simulink model "model"  (R2016a)
(part 11 of 11)

  _CN_176704629_220000_CN30425117/RConn3 -- G_30425117_Kraftwerk_Weiher/RConn3 -- _CN_54359256_220000_CN30425117/RConn3 -- _CN_100812630_220000_CN30425117/LConn3
  T_150267232_220000_LMG/LConn1 -- 220kV_LMG_West_CN_24921206_220000_CN_150267232_220000/RConn1
  T_150267232_220000_LMG/LConn2 -- 220kV_LMG_West_CN_24921206_220000_CN_150267232_220000/RConn2
  T_150267232_220000_LMG/LConn3 -- 220kV_LMG_West_CN_24921206_220000_CN_150267232_220000/RConn3
  T_42423415_220000;110000_Station_Meckenheim/LConn1 -- 220_kV_Berggeist_West;_Nette_Ost_CN_42423415_220000_CN_395847307_220000/RConn1
  T_42423415_220000;110000_Station_Meckenheim/LConn2 -- 220_kV_Berggeist_West;_Nette_Ost_CN_42423415_220000_CN_395847307_220000/RConn2
  T_42423415_220000;110000_Station_Meckenheim/LConn3 -- 220_kV_Berggeist_West;_Nette_Ost_CN_42423415_220000_CN_395847307_220000/RConn3
  _CN_42681484_380000_CN_274630377_380000/LConn1 -- T_42681484_380000;110000_Vörden/LConn1 -- _CN_42681484_380000_CN_24413992_380000/RConn1
  _CN_42681484_380000_CN_274630377_380000/LConn2 -- T_42681484_380000;110000_Vörden/LConn2 -- _CN_42681484_380000_CN_24413992_380000/RConn2
  _CN_42681484_380000_CN_274630377_380000/LConn3 -- T_42681484_380000;110000_Vörden/LConn3 -- _CN_42681484_380000_CN_24413992_380000/RConn3
  _CN_42681484_380000_CN_274630377_380000/RConn1 -- T_274630377_380000;220000;110000_Umspannanlage_Würgassen/LConn1 -- _CN_274630377_380000_CN_156960655_380000/LConn1
  _CN_42681484_380000_CN_274630377_380000/RConn2 -- T_274630377_380000;220000;110000_Umspannanlage_Würgassen/LConn2 -- _CN_274630377_380000_CN_156960655_380000/LConn2
  _CN_42681484_380000_CN_274630377_380000/RConn3 -- T_274630377_380000;220000;110000_Umspannanlage_Würgassen/LConn3 -- _CN_274630377_380000_CN_156960655_380000/LConn3
  _CN_128277645_220000_CN_152219167_220000/LConn1 -- T_128277645_380000;220000;110000_Umspannwerk_Remptendorf/RConn1 -- _CN_128277645_220000_CN136858836/LConn1
  _CN_128277645_220000_CN_152219167_220000/LConn2 -- T_128277645_380000;220000;110000_Umspannwerk_Remptendorf/RConn2 -- _CN_128277645_220000_CN136858836/LConn2
  _CN_128277645_220000_CN_152219167_220000/LConn3 -- T_128277645_380000;220000;110000_Umspannwerk_Remptendorf/RConn3 -- _CN_128277645_220000_CN136858836/LConn3
  T_152219167_220000_Stahlwerk_Thüringen/LConn1 -- _CN_128277645_220000_CN_152219167_220000/RConn1
  T_152219167_220000_Stahlwerk_Thüringen/LConn2 -- _CN_128277645_220000_CN_152219167_220000/RConn2
  T_152219167_220000_Stahlwerk_Thüringen/LConn3 -- _CN_128277645_220000_CN_152219167_220000/RConn3
  G_136858836_Pumpspeicherkraftwerk_Hohenwarte_II/RConn1 -- _CN_128277645_220000_CN136858836/RConn1
  G_136858836_Pumpspeicherkraftwerk_Hohenwarte_II/RConn2 -- _CN_128277645_220000_CN136858836/RConn2
  G_136858836_Pumpspeicherkraftwerk_Hohenwarte_II/RConn3 -- _CN_128277645_220000_CN136858836/RConn3
  T_156673637_380000;220000;110000_Umspannwerk_Weida/LConn1 -- 574_Remptendorf___Röhrsdorf;_573_Remptendorf___Weida_CN_128277645_380000_CN_156673637_380000/RConn1
  T_156673637_380000;220000;110000_Umspannwerk_Weida/LConn2 -- 574_Remptendorf___Röhrsdorf;_573_Remptendorf___Weida_CN_128277645_380000_CN_156673637_380000/RConn2
  T_156673637_380000;220000;110000_Umspannwerk_Weida/LConn3 -- 574_Remptendorf___Röhrsdorf;_573_Remptendorf___Weida_CN_128277645_380000_CN_156673637_380000/RConn3
  _CN_24536211_380000_CN_202747445_380000/RConn1 -- T_24536211_380000;110000_Umspannwerk_Aßlar/LConn1 -- _CN_24536211_380000_CN_152403632_380000/RConn1 -- _CN_24536211_380000_CN_24536328_380000/LConn1
  _CN_24536211_380000_CN_202747445_380000/RConn2 -- T_24536211_380000;110000_Umspannwerk_Aßlar/LConn2 -- _CN_24536211_380000_CN_152403632_380000/RConn2 -- _CN_24536211_380000_CN_24536328_380000/LConn2
  _CN_24536211_380000_CN_202747445_380000/RConn3 -- T_24536211_380000;110000_Umspannwerk_Aßlar/LConn3 -- _CN_24536211_380000_CN_152403632_380000/RConn3 -- _CN_24536211_380000_CN_24536328_380000/LConn3
  T_24536328_380000;110000_Dillenburg/LConn1 -- _CN_24536211_380000_CN_24536328_380000/RConn1
  T_24536328_380000;110000_Dillenburg/LConn2 -- _CN_24536211_380000_CN_24536328_380000/RConn2
  T_24536328_380000;110000_Dillenburg/LConn3 -- _CN_24536211_380000_CN_24536328_380000/RConn3
  T_23161029_220000;110000_Umspannwerk_Taucha/LConn1 -- _CN_23161029_220000_CN_32843531_220000/LConn1
  T_23161029_220000;110000_Umspannwerk_Taucha/LConn2 -- _CN_23161029_220000_CN_32843531_220000/LConn2
  T_23161029_220000;110000_Umspannwerk_Taucha/LConn3 -- _CN_23161029_220000_CN_32843531_220000/LConn3
  _CN_23161029_220000_CN_32843531_220000/RConn1 -- T_32843531_380000;220000;110000_Eula/RConn1 -- _CN_22879599_220000_CN_32843531_220000/RConn1 -- 203_Eula_CN_23117075_220000_CN_32843531_220000/RConn1
  _CN_23161029_220000_CN_32843531_220000/RConn2 -- T_32843531_380000;220000;110000_Eula/RConn2 -- _CN_22879599_220000_CN_32843531_220000/RConn2 -- 203_Eula_CN_23117075_220000_CN_32843531_220000/RConn2
  _CN_23161029_220000_CN_32843531_220000/RConn3 -- T_32843531_380000;220000;110000_Eula/RConn3 -- _CN_22879599_220000_CN_32843531_220000/RConn3 -- 203_Eula_CN_23117075_220000_CN_32843531_220000/RConn3
  T_201153704_380000;220000_Kraftwerkschaltanlage_Knapsack_1/LConn1 -- 380_kV_Knapsack_1a_CN_201153704_380000_CN_22765517_380000/RConn1
  T_201153704_380000;220000_Kraftwerkschaltanlage_Knapsack_1/LConn2 -- 380_kV_Knapsack_1a_CN_201153704_380000_CN_22765517_380000/RConn2
  T_201153704_380000;220000_Kraftwerkschaltanlage_Knapsack_1/LConn3 -- 380_kV_Knapsack_1a_CN_201153704_380000_CN_22765517_380000/RConn3
  T_24478889_220000;110000_Station_Walsum/LConn1 -- 220kV_Beeck_Tr211+212_CN_24478889_220000_CN26623135/RConn1
  T_24478889_220000;110000_Station_Walsum/LConn2 -- 220kV_Beeck_Tr211+212_CN_24478889_220000_CN26623135/RConn2
  T_24478889_220000;110000_Station_Walsum/LConn3 -- 220kV_Beeck_Tr211+212_CN_24478889_220000_CN26623135/RConn3
  380_kV_Transversale_Berlin_CN_46615737_380000_CN_30303506_380000/RConn1 -- T_30303506_380000;110000_Berlin_Mitte/LConn1 -- 380_kV_Transversale_Berlin_CN_30954714_380000_CN_30303506_380000/RConn1
  380_kV_Transversale_Berlin_CN_46615737_380000_CN_30303506_380000/RConn2 -- T_30303506_380000;110000_Berlin_Mitte/LConn2 -- 380_kV_Transversale_Berlin_CN_30954714_380000_CN_30303506_380000/RConn2
  380_kV_Transversale_Berlin_CN_46615737_380000_CN_30303506_380000/RConn3 -- T_30303506_380000;110000_Berlin_Mitte/LConn3 -- 380_kV_Transversale_Berlin_CN_30954714_380000_CN_30303506_380000/RConn3
  T_83916207_220000;110000_Elverlingsen/LConn1 -- 220kV_Nordleitung_CN_24667346_220000_CN_83916207_220000/RConn1
  T_83916207_220000;110000_Elverlingsen/LConn2 -- 220kV_Nordleitung_CN_24667346_220000_CN_83916207_220000/RConn2
  T_83916207_220000;110000_Elverlingsen/LConn3 -- 220kV_Nordleitung_CN_24667346_220000_CN_83916207_220000/RConn3
  _CN_54359256_380000_CN115145869/RConn1 -- G_115145869_Kraftwerk_Ensdorf/RConn1 -- 220_kV_CN_82773910_220000_CN115145869/LConn1 -- _CN_82773910_380000_CN115145869/LConn1
  _CN_54359256_380000_CN115145869/RConn2 -- G_115145869_Kraftwerk_Ensdorf/RConn2 -- 220_kV_CN_82773910_220000_CN115145869/LConn2 -- _CN_82773910_380000_CN115145869/LConn2
  _CN_54359256_380000_CN115145869/RConn3 -- G_115145869_Kraftwerk_Ensdorf/RConn3 -- 220_kV_CN_82773910_220000_CN115145869/LConn3 -- _CN_82773910_380000_CN115145869/LConn3
  _CN_54359256_220000_CN_100812630_220000/RConn1 -- T_100812630_220000;110000_/LConn1 -- _CN_100812630_220000_CN30425117/RConn1
  _CN_54359256_220000_CN_100812630_220000/RConn2 -- T_100812630_220000;110000_/LConn2 -- _CN_100812630_220000_CN30425117/RConn2
  _CN_54359256_220000_CN_100812630_220000/RConn3 -- T_100812630_220000;110000_/LConn3 -- _CN_100812630_220000_CN30425117/RConn3
  G_58421134_Kraftwerk_Schwarze_Pumpe/RConn1 -- _CN_30164703_380000_CN58421134/RConn1
  G_58421134_Kraftwerk_Schwarze_Pumpe/RConn2 -- _CN_30164703_380000_CN58421134/RConn2
  G_58421134_Kraftwerk_Schwarze_Pumpe/RConn3 -- _CN_30164703_380000_CN58421134/RConn3
  T_30309989_220000_Hennigsdorf/LConn1 -- 294_CN_27149550_220000_CN_30309989_220000/RConn1
  T_30309989_220000_Hennigsdorf/LConn2 -- 294_CN_27149550_220000_CN_30309989_220000/RConn2
  T_30309989_220000_Hennigsdorf/LConn3 -- 294_CN_27149550_220000_CN_30309989_220000/RConn3
  G_101400025_Kraftwerk_Moorburg/RConn1 -- _CN_11285720_380000_CN101400025/RConn1
  G_101400025_Kraftwerk_Moorburg/RConn2 -- _CN_11285720_380000_CN101400025/RConn2
  G_101400025_Kraftwerk_Moorburg/RConn3 -- _CN_11285720_380000_CN101400025/RConn3
  T_35763481_380000;110000_Station_Witten/LConn1 -- Trafo_411_CN_35763480_380000_CN_35763481_380000/RConn1
  T_35763481_380000;110000_Station_Witten/LConn2 -- Trafo_411_CN_35763480_380000_CN_35763481_380000/RConn2
  T_35763481_380000;110000_Station_Witten/LConn3 -- Trafo_411_CN_35763480_380000_CN_35763481_380000/RConn3
  T_24479003_220000_Station_Möllen/LConn1 -- _CN_24479003_380000_CN401873466/RConn1
  T_24479003_220000_Station_Möllen/LConn2 -- _CN_24479003_380000_CN401873466/RConn2
  T_24479003_220000_Station_Möllen/LConn3 -- _CN_24479003_380000_CN401873466/RConn3
  T_24479003_220000_Station_Möllen/RConn1 -- _CN_24479003_220000_CN401873466/RConn1
  T_24479003_220000_Station_Möllen/RConn2 -- _CN_24479003_220000_CN401873466/RConn2
  T_24479003_220000_Station_Möllen/RConn3 -- _CN_24479003_220000_CN401873466/RConn3
  220kV_Gersteinwerk_I2_CN_42507488_220000_CN33883956/RConn1 -- G_33883956_/RConn1 -- 380kV_Gersteinwerk_K2_CN_42507488_380000_CN33883956/RConn1
  220kV_Gersteinwerk_I2_CN_42507488_220000_CN33883956/RConn2 -- G_33883956_/RConn2 -- 380kV_Gersteinwerk_K2_CN_42507488_380000_CN33883956/RConn2
  220kV_Gersteinwerk_I2_CN_42507488_220000_CN33883956/RConn3 -- G_33883956_/RConn3 -- 380kV_Gersteinwerk_K2_CN_42507488_380000_CN33883956/RConn3
  G_88700172_Gersteinwerk_Block_F/RConn1 -- 220kV_Gersteinwerk_F2_CN_42507488_220000_CN88700172/RConn1
  G_88700172_Gersteinwerk_Block_F/RConn2 -- 220kV_Gersteinwerk_F2_CN_42507488_220000_CN88700172/RConn2
  G_88700172_Gersteinwerk_Block_F/RConn3 -- 220kV_Gersteinwerk_F2_CN_42507488_220000_CN88700172/RConn3
  T_29420322_220000;155000_Inhausen/LConn1 -- 211_CN_29420322_220000_CN_26455019_220000/LConn1
  T_29420322_220000;155000_Inhausen/LConn2 -- 211_CN_29420322_220000_CN_26455019_220000/LConn2
  T_29420322_220000;155000_Inhausen/LConn3 -- 211_CN_29420322_220000_CN_26455019_220000/LConn3
  211_CN_29420322_220000_CN_26455019_220000/RConn1 -- T_26455019_220000;110000_Voslapp/LConn1 -- Voslapp_CN_23744346_220000_CN_26455019_220000/LConn1
  211_CN_29420322_220000_CN_26455019_220000/RConn2 -- T_26455019_220000;110000_Voslapp/LConn2 -- Voslapp_CN_23744346_220000_CN_26455019_220000/LConn2
  211_CN_29420322_220000_CN_26455019_220000/RConn3 -- T_26455019_220000;110000_Voslapp/LConn3 -- Voslapp_CN_23744346_220000_CN_26455019_220000/LConn3
  T_48428875_380000;110000_EnBW_Umspannwerk_Endersbach/LConn1 -- AL1_EDS_380_kV_CN_48428875_380000_CN25973419/RConn1
  T_48428875_380000;110000_EnBW_Umspannwerk_Endersbach/LConn2 -- AL1_EDS_380_kV_CN_48428875_380000_CN25973419/RConn2
  T_48428875_380000;110000_EnBW_Umspannwerk_Endersbach/LConn3 -- AL1_EDS_380_kV_CN_48428875_380000_CN25973419/RConn3
  T_156676050_220000;110000_Umspannanlage_Heidelberg_Süd/LConn1 -- _CN_207248812_220000_CN_156676050_220000/RConn1
  T_156676050_220000;110000_Umspannanlage_Heidelberg_Süd/LConn2 -- _CN_207248812_220000_CN_156676050_220000/RConn2
  T_156676050_220000;110000_Umspannanlage_Heidelberg_Süd/LConn3 -- _CN_207248812_220000_CN_156676050_220000/RConn3
  T_87952821_380000;220000;110000;20000_Flensburg/RConn1 -- _CN_87952821_220000_CN_33148774_220000/RConn1
  T_87952821_380000;220000;110000;20000_Flensburg/RConn2 -- _CN_87952821_220000_CN_33148774_220000/RConn2
  T_87952821_380000;220000;110000;20000_Flensburg/RConn3 -- _CN_87952821_220000_CN_33148774_220000/RConn3
  380kV_Voerde_B_CN_76185022_380000_CN401873466/RConn1 -- T_76185022_380000_Station_Zensenbusch/LConn1 -- _CN_76185022_380000_CN26623135/RConn1
  380kV_Voerde_B_CN_76185022_380000_CN401873466/RConn2 -- T_76185022_380000_Station_Zensenbusch/LConn2 -- _CN_76185022_380000_CN26623135/RConn2
  380kV_Voerde_B_CN_76185022_380000_CN401873466/RConn3 -- T_76185022_380000_Station_Zensenbusch/LConn3 -- _CN_76185022_380000_CN26623135/RConn3
  T_37721677_380000;110000_EnBW_Umspannwerk_Altbach_1/LConn1 -- AL1_BZW_380_kV_CN_37721677_380000_CN25973419/RConn1
  T_37721677_380000;110000_EnBW_Umspannwerk_Altbach_1/LConn2 -- AL1_BZW_380_kV_CN_37721677_380000_CN25973419/RConn2
  T_37721677_380000;110000_EnBW_Umspannwerk_Altbach_1/LConn3 -- AL1_BZW_380_kV_CN_37721677_380000_CN25973419/RConn3
  G_218161891_Kraftwerk_Schkopau/RConn1 -- _CN_29713902_380000_CN218161891/RConn1
  G_218161891_Kraftwerk_Schkopau/RConn2 -- _CN_29713902_380000_CN218161891/RConn2
  G_218161891_Kraftwerk_Schkopau/RConn3 -- _CN_29713902_380000_CN218161891/RConn3
  T_43163132_380000;110000_Umspannwerk_Reuter/LConn1 -- _CN_43163132_380000_CN185569568/RConn1
  T_43163132_380000;110000_Umspannwerk_Reuter/LConn2 -- _CN_43163132_380000_CN185569568/RConn2
  T_43163132_380000;110000_Umspannwerk_Reuter/LConn3 -- _CN_43163132_380000_CN185569568/RConn3
  T_154869247_220000_/LConn1 -- _CN_154869247_220000_CN_395847307_220000/RConn1
  T_154869247_220000_/LConn2 -- _CN_154869247_220000_CN_395847307_220000/RConn2
  T_154869247_220000_/LConn3 -- _CN_154869247_220000_CN_395847307_220000/RConn3
  Leitung_2008_CN_28921360_220000_CN-2022229/RConn1 -- T_28921360_220000_Umspannwerk_Kraftwerk_Robert_Frank/LConn1 -- Leitung_3004_CN_28921360_220000_CN_27739871_220000/LConn1
  Leitung_2008_CN_28921360_220000_CN-2022229/RConn2 -- T_28921360_220000_Umspannwerk_Kraftwerk_Robert_Frank/LConn2 -- Leitung_3004_CN_28921360_220000_CN_27739871_220000/LConn2
  Leitung_2008_CN_28921360_220000_CN-2022229/RConn3 -- T_28921360_220000_Umspannwerk_Kraftwerk_Robert_Frank/LConn3 -- Leitung_3004_CN_28921360_220000_CN_27739871_220000/LConn3
  Leitung_3004_CN_28921360_220000_CN_27739871_220000/RConn1 -- T_27739871_380000;220000_Landesbergen/RConn1 -- L_27739871/LConn1
  Leitung_3004_CN_28921360_220000_CN_27739871_220000/RConn2 -- T_27739871_380000;220000_Landesbergen/RConn2 -- L_27739871/LConn2
  Leitung_3004_CN_28921360_220000_CN_27739871_220000/RConn3 -- T_27739871_380000;220000_Landesbergen/RConn3 -- L_27739871/LConn3
  Dellmensingen___Obermooweiler;Dellmensingen_Ost_CN_41389594_380000_CN_31131320_380000/RConn1 -- T_31131320_380000_Umspannwerk_Obermooweiler/LConn1 -- _CN_31131320_380000_CN_31131325_380000/RConn1
  Dellmensingen___Obermooweiler;Dellmensingen_Ost_CN_41389594_380000_CN_31131320_380000/RConn2 -- T_31131320_380000_Umspannwerk_Obermooweiler/LConn2 -- _CN_31131320_380000_CN_31131325_380000/RConn2
  Dellmensingen___Obermooweiler;Dellmensingen_Ost_CN_41389594_380000_CN_31131320_380000/RConn3 -- T_31131320_380000_Umspannwerk_Obermooweiler/LConn3 -- _CN_31131320_380000_CN_31131325_380000/RConn3
  T_97857512_220000_/LConn1 -- _CN_28227099_220000_CN_97857512_220000/RConn1
  T_97857512_220000_/LConn2 -- _CN_28227099_220000_CN_97857512_220000/RConn2
  T_97857512_220000_/LConn3 -- _CN_28227099_220000_CN_97857512_220000/RConn3
  T_42872354_220000_Huntorf/LConn1 -- Huntorf_CN_42872354_220000_CN42872353/LConn1
  T_42872354_220000_Huntorf/LConn2 -- Huntorf_CN_42872354_220000_CN42872353/LConn2
  T_42872354_220000_Huntorf/LConn3 -- Huntorf_CN_42872354_220000_CN42872353/LConn3
  G_42872353_Druckluftspeicher__und_Gasturbinenkraftwerk_Huntorf/RConn1 -- Huntorf_CN_42872354_220000_CN42872353/RConn1
  G_42872353_Druckluftspeicher__und_Gasturbinenkraftwerk_Huntorf/RConn2 -- Huntorf_CN_42872354_220000_CN42872353/RConn2
  G_42872353_Druckluftspeicher__und_Gasturbinenkraftwerk_Huntorf/RConn3 -- Huntorf_CN_42872354_220000_CN42872353/RConn3
  _CN_23881272_220000_CN145861680/RConn1 -- T_23881272_220000;110000_Dörnigheim_220_kV/LConn1 -- _CN_23881272_220000_CN_4826893_220000/LConn1
  _CN_23881272_220000_CN145861680/RConn2 -- T_23881272_220000;110000_Dörnigheim_220_kV/LConn2 -- _CN_23881272_220000_CN_4826893_220000/LConn2
  _CN_23881272_220000_CN145861680/RConn3 -- T_23881272_220000;110000_Dörnigheim_220_kV/LConn3 -- _CN_23881272_220000_CN_4826893_220000/LConn3
  T_4826893_220000;110000_Umspannwerk_Frankfurt_Nord/LConn1 -- _CN_23881272_220000_CN_4826893_220000/RConn1
  T_4826893_220000;110000_Umspannwerk_Frankfurt_Nord/LConn2 -- _CN_23881272_220000_CN_4826893_220000/RConn2
  T_4826893_220000;110000_Umspannwerk_Frankfurt_Nord/LConn3 -- _CN_23881272_220000_CN_4826893_220000/RConn3
  T_32675761_380000;110000_Station_Dahlem/LConn1 -- _CN_151967290_380000_CN_32675761_380000/RConn1
  T_32675761_380000;110000_Station_Dahlem/LConn2 -- _CN_151967290_380000_CN_32675761_380000/RConn2
  T_32675761_380000;110000_Station_Dahlem/LConn3 -- _CN_151967290_380000_CN_32675761_380000/RConn3
  T_167352587_220000;110000_Umspannwerk_Herlasgrün/LConn1 -- 231;_232_Weida___Herlasgrün_CN_167352587_220000_CN_156673637_220000/LConn1
  T_167352587_220000;110000_Umspannwerk_Herlasgrün/LConn2 -- 231;_232_Weida___Herlasgrün_CN_167352587_220000_CN_156673637_220000/LConn2
  T_167352587_220000;110000_Umspannwerk_Herlasgrün/LConn3 -- 231;_232_Weida___Herlasgrün_CN_167352587_220000_CN_156673637_220000/LConn3
  T_156673637_380000;220000;110000_Umspannwerk_Weida/RConn1 -- 231;_232_Weida___Herlasgrün_CN_167352587_220000_CN_156673637_220000/RConn1
  T_156673637_380000;220000;110000_Umspannwerk_Weida/RConn2 -- 231;_232_Weida___Herlasgrün_CN_167352587_220000_CN_156673637_220000/RConn2
  T_156673637_380000;220000;110000_Umspannwerk_Weida/RConn3 -- 231;_232_Weida___Herlasgrün_CN_167352587_220000_CN_156673637_220000/RConn3
  G_109373271_RWE_Kraftwerk_Neurath_BoA_Bl__F_G/RConn1 -- 380_kV_Neurath_4d|5e_CN_207488608_380000_CN109373271/RConn1
  G_109373271_RWE_Kraftwerk_Neurath_BoA_Bl__F_G/RConn2 -- 380_kV_Neurath_4d|5e_CN_207488608_380000_CN109373271/RConn2
  G_109373271_RWE_Kraftwerk_Neurath_BoA_Bl__F_G/RConn3 -- 380_kV_Neurath_4d|5e_CN_207488608_380000_CN109373271/RConn3
  G_125808869_Kraftwerk_Hamborn_Block_5/RConn1 -- _CN_35833442_220000_CN125808869/RConn1
  G_125808869_Kraftwerk_Hamborn_Block_5/RConn2 -- _CN_35833442_220000_CN125808869/RConn2
  G_125808869_Kraftwerk_Hamborn_Block_5/RConn3 -- _CN_35833442_220000_CN125808869/RConn3
  _CN_156673636_380000_CN_156960655_380000/RConn1 -- T_156960655_380000;110000_Umspannwerk_Bergshausen/LConn1 -- _CN_274630377_380000_CN_156960655_380000/RConn1
  _CN_156673636_380000_CN_156960655_380000/RConn2 -- T_156960655_380000;110000_Umspannwerk_Bergshausen/LConn2 -- _CN_274630377_380000_CN_156960655_380000/RConn2
  _CN_156673636_380000_CN_156960655_380000/RConn3 -- T_156960655_380000;110000_Umspannwerk_Bergshausen/LConn3 -- _CN_274630377_380000_CN_156960655_380000/RConn3
  T_41072584_380000_UW_Waldeck/LConn1 -- Leitung_3212;Leitung_3213_CN_156673636_380000_CN_41072584_380000/RConn1
  T_41072584_380000_UW_Waldeck/LConn2 -- Leitung_3212;Leitung_3213_CN_156673636_380000_CN_41072584_380000/RConn2
  T_41072584_380000_UW_Waldeck/LConn3 -- Leitung_3212;Leitung_3213_CN_156673636_380000_CN_41072584_380000/RConn3
  T_106976898_220000_Saarstahl/LConn1 -- _CN_106976898_220000_CN_31135714_220000/LConn1
  T_106976898_220000_Saarstahl/LConn2 -- _CN_106976898_220000_CN_31135714_220000/LConn2
  T_106976898_220000_Saarstahl/LConn3 -- _CN_106976898_220000_CN_31135714_220000/LConn3
  T_31135714_220000;110000_Umspannwerk_Heinitz/LConn1 -- _CN_106976898_220000_CN_31135714_220000/RConn1
  T_31135714_220000;110000_Umspannwerk_Heinitz/LConn2 -- _CN_106976898_220000_CN_31135714_220000/RConn2
  T_31135714_220000;110000_Umspannwerk_Heinitz/LConn3 -- _CN_106976898_220000_CN_31135714_220000/RConn3
  T_25992879_380000;110000_Siersdorf/LConn1 -- _CN_25992879_380000_CN_26593929_380000/RConn1
  T_25992879_380000;110000_Siersdorf/LConn2 -- _CN_25992879_380000_CN_26593929_380000/RConn2
  T_25992879_380000;110000_Siersdorf/LConn3 -- _CN_25992879_380000_CN_26593929_380000/RConn3
  204_CN_173178563_220000_CN_23744346_220000/RConn1 -- T_23744346_380000;220000_Umspannwerk_Maade/LConn1 -- 300_CN_23744346_220000_CN26470129/LConn1 -- Voslapp_CN_23744346_220000_CN_26455019_220000/RConn1 -- Maade_gelb_CN_157421330_220000_CN_23744346_220000/LConn1
  204_CN_173178563_220000_CN_23744346_220000/RConn2 -- T_23744346_380000;220000_Umspannwerk_Maade/LConn2 -- 300_CN_23744346_220000_CN26470129/LConn2 -- Voslapp_CN_23744346_220000_CN_26455019_220000/RConn2 -- Maade_gelb_CN_157421330_220000_CN_23744346_220000/LConn2
  204_CN_173178563_220000_CN_23744346_220000/RConn3 -- T_23744346_380000;220000_Umspannwerk_Maade/LConn3 -- 300_CN_23744346_220000_CN26470129/LConn3 -- Voslapp_CN_23744346_220000_CN_26455019_220000/RConn3 -- Maade_gelb_CN_157421330_220000_CN_23744346_220000/LConn3
  G_150031354_/RConn1 -- _CN_27739871_380000_CN150031354/RConn1
  G_150031354_/RConn2 -- _CN_27739871_380000_CN150031354/RConn2
  G_150031354_/RConn3 -- _CN_27739871_380000_CN150031354/RConn3
  T_157449983_380000_/LConn1 -- Emsland_D1|D2|D0_CN_157449983_380000_CN49339874/RConn1
  T_157449983_380000_/LConn2 -- Emsland_D1|D2|D0_CN_157449983_380000_CN49339874/RConn2
  T_157449983_380000_/LConn3 -- Emsland_D1|D2|D0_CN_157449983_380000_CN49339874/RConn3
  T_157421330_220000_Atlantic/LConn1 -- Maade_gelb_CN_157421330_220000_CN_23744346_220000/RConn1
  T_157421330_220000_Atlantic/LConn2 -- Maade_gelb_CN_157421330_220000_CN_23744346_220000/RConn2
  T_157421330_220000_Atlantic/LConn3 -- Maade_gelb_CN_157421330_220000_CN_23744346_220000/RConn3
  G_26470129_Uniper_Kraftwerk_Wilhelmshaven/RConn1 -- 300_CN_23744346_220000_CN26470129/RConn1
  G_26470129_Uniper_Kraftwerk_Wilhelmshaven/RConn2 -- 300_CN_23744346_220000_CN26470129/RConn2
  G_26470129_Uniper_Kraftwerk_Wilhelmshaven/RConn3 -- 300_CN_23744346_220000_CN26470129/RConn3
  T_82773910_380000;220000;110000_Umspannanlage_Ensdorf/RConn1 -- 220_kV_CN_82773910_220000_CN115145869/RConn1
  T_82773910_380000;220000;110000_Umspannanlage_Ensdorf/RConn2 -- 220_kV_CN_82773910_220000_CN115145869/RConn2
  T_82773910_380000;220000;110000_Umspannanlage_Ensdorf/RConn3 -- 220_kV_CN_82773910_220000_CN115145869/RConn3
  T_82773910_380000;220000;110000_Umspannanlage_Ensdorf/LConn1 -- _CN_82773910_380000_CN115145869/RConn1
  T_82773910_380000;220000;110000_Umspannanlage_Ensdorf/LConn2 -- _CN_82773910_380000_CN115145869/RConn2
  T_82773910_380000;220000;110000_Umspannanlage_Ensdorf/LConn3 -- _CN_82773910_380000_CN115145869/RConn3
  G_-536706_Kraftwerk_Knepper/RConn1 -- 220kV_Knepper_C_CN_28452784_220000_CN-536706/RConn1
  G_-536706_Kraftwerk_Knepper/RConn2 -- 220kV_Knepper_C_CN_28452784_220000_CN-536706/RConn2
  G_-536706_Kraftwerk_Knepper/RConn3 -- 220kV_Knepper_C_CN_28452784_220000_CN-536706/RConn3
  T_42411962_220000;110000_Kraftwerkseinspeisung_Staudinger/LConn1 -- _CN_42411962_220000_CN145861680/RConn1
  T_42411962_220000;110000_Kraftwerkseinspeisung_Staudinger/LConn2 -- _CN_42411962_220000_CN145861680/RConn2
  T_42411962_220000;110000_Kraftwerkseinspeisung_Staudinger/LConn3 -- _CN_42411962_220000_CN145861680/RConn3
  G_11341038_Kraftwerk_Jänschwalde/RConn1 -- _CN_23025610_380000_CN11341038/RConn1
  G_11341038_Kraftwerk_Jänschwalde/RConn2 -- _CN_23025610_380000_CN11341038/RConn2
  G_11341038_Kraftwerk_Jänschwalde/RConn3 -- _CN_23025610_380000_CN11341038/RConn3
  T_23816140_220000;110000_Lahe/LConn1 -- _CN_23816140_220000_CN23681460/RConn1
  T_23816140_220000;110000_Lahe/LConn2 -- _CN_23816140_220000_CN23681460/RConn2
  T_23816140_220000;110000_Lahe/LConn3 -- _CN_23816140_220000_CN23681460/RConn3
  G_239364386_Statkraft_Kraftwerk_Knapsack_II/RConn1 -- _CN_22765517_380000_CN239364386/RConn1
  G_239364386_Statkraft_Kraftwerk_Knapsack_II/RConn2 -- _CN_22765517_380000_CN239364386/RConn2
  G_239364386_Statkraft_Kraftwerk_Knapsack_II/RConn3 -- _CN_22765517_380000_CN239364386/RConn3
  T_275138524_380000;110000_Schaltanlage_Datteln_4/LConn1 -- _CN_275138524_380000_CN109504648/RConn1
  T_275138524_380000;110000_Schaltanlage_Datteln_4/LConn2 -- _CN_275138524_380000_CN109504648/RConn2
  T_275138524_380000;110000_Schaltanlage_Datteln_4/LConn3 -- _CN_275138524_380000_CN109504648/RConn3
  T_24258096_380000_Umspannwerk_Hattorf/RConn1 -- L_24258096/LConn1
  T_24258096_380000_Umspannwerk_Hattorf/RConn2 -- L_24258096/LConn2
  T_24258096_380000_Umspannwerk_Hattorf/RConn3 -- L_24258096/LConn3
  T_30017786_220000_Gleidingen_220_kV/RConn1 -- L_30017786/LConn1
  T_30017786_220000_Gleidingen_220_kV/RConn2 -- L_30017786/LConn2
  T_30017786_220000_Gleidingen_220_kV/RConn3 -- L_30017786/LConn3
  T_28227099_220000;110000_Salzgitter_Hallendorf/RConn1 -- L_28227099/LConn1
  T_28227099_220000;110000_Salzgitter_Hallendorf/RConn2 -- L_28227099/LConn2
  T_28227099_220000;110000_Salzgitter_Hallendorf/RConn3 -- L_28227099/LConn3
  T_23899043_380000;110000_Algermissen/RConn1 -- L_23899043/LConn1
  T_23899043_380000;110000_Algermissen/RConn2 -- L_23899043/LConn2
  T_23899043_380000;110000_Algermissen/RConn3 -- L_23899043/LConn3
  T_24413992_380000;110000_UW_Grohnde_380_kV___110_kV/RConn1 -- L_24413992/LConn1
  T_24413992_380000;110000_UW_Grohnde_380_kV___110_kV/RConn2 -- L_24413992/LConn2
  T_24413992_380000;110000_UW_Grohnde_380_kV___110_kV/RConn3 -- L_24413992/LConn3
  T_24272339_380000;110000_Klein_Ilsede/RConn1 -- L_24272339/LConn1
  T_24272339_380000;110000_Klein_Ilsede/RConn2 -- L_24272339/LConn2
  T_24272339_380000;110000_Klein_Ilsede/RConn3 -- L_24272339/LConn3
  T_24272541_220000_Umspannwerk_Braunschweig_Nord/RConn1 -- L_24272541/LConn1
  T_24272541_220000_Umspannwerk_Braunschweig_Nord/RConn2 -- L_24272541/LConn2
  T_24272541_220000_Umspannwerk_Braunschweig_Nord/RConn3 -- L_24272541/LConn3
  T_28343121_380000_Stadorf/RConn1 -- L_28343121/LConn1
  T_28343121_380000_Stadorf/RConn2 -- L_28343121/LConn2
  T_28343121_380000_Stadorf/RConn3 -- L_28343121/LConn3
  T_24415232_220000;110000_Station_Elmenhorst/RConn1 -- L_24415232/LConn1
  T_24415232_220000;110000_Station_Elmenhorst/RConn2 -- L_24415232/LConn2
  T_24415232_220000;110000_Station_Elmenhorst/RConn3 -- L_24415232/LConn3
  T_28452784_220000;110000_Station_Pöppinghausen/RConn1 -- L_28452784/LConn1
  T_28452784_220000;110000_Station_Pöppinghausen/RConn2 -- L_28452784/LConn2
  T_28452784_220000;110000_Station_Pöppinghausen/RConn3 -- L_28452784/LConn3
  T_138877959_220000_Rheinzink/RConn1 -- L_138877959/LConn1
  T_138877959_220000_Rheinzink/RConn2 -- L_138877959/LConn2
  T_138877959_220000_Rheinzink/RConn3 -- L_138877959/LConn3
  T_42507488_380000;220000;110000_Station_Gersteinwerk/RConn4 -- L_42507488/LConn1
  T_42507488_380000;220000;110000_Station_Gersteinwerk/RConn5 -- L_42507488/LConn2
  T_42507488_380000;220000;110000_Station_Gersteinwerk/RConn6 -- L_42507488/LConn3
  T_41334805_220000_Drehstromschaltwerk_Neckarwestheim/RConn1 -- L_41334805/LConn1
  T_41334805_220000_Drehstromschaltwerk_Neckarwestheim/RConn2 -- L_41334805/LConn2
  T_41334805_220000_Drehstromschaltwerk_Neckarwestheim/RConn3 -- L_41334805/LConn3
  T_25786404_220000;110000_Umspannwerk_Hoheneck_EnBW/RConn1 -- L_25786404/LConn1
  T_25786404_220000;110000_Umspannwerk_Hoheneck_EnBW/RConn2 -- L_25786404/LConn2
  T_25786404_220000;110000_Umspannwerk_Hoheneck_EnBW/RConn3 -- L_25786404/LConn3
  T_43688805_380000;220000;110000_380kV_Umspannwerk_Pulverdingen/RConn4 -- L_43688805/LConn1
  T_43688805_380000;220000;110000_380kV_Umspannwerk_Pulverdingen/RConn5 -- L_43688805/LConn2
  T_43688805_380000;220000;110000_380kV_Umspannwerk_Pulverdingen/RConn6 -- L_43688805/LConn3
  T_23414063_220000;110000_Umspannwerk_Weilimdorf/RConn1 -- L_23414063/LConn1
  T_23414063_220000;110000_Umspannwerk_Weilimdorf/RConn2 -- L_23414063/LConn2
  T_23414063_220000;110000_Umspannwerk_Weilimdorf/RConn3 -- L_23414063/LConn3
  T_143903369_380000;220000;110000_Umspannwerk_Hüffenhardt/RConn4 -- L_143903369/LConn1
  T_143903369_380000;220000;110000_Umspannwerk_Hüffenhardt/RConn5 -- L_143903369/LConn2
  T_143903369_380000;220000;110000_Umspannwerk_Hüffenhardt/RConn6 -- L_143903369/LConn3
  T_152973139_220000;110000_Station_Rheinau/RConn1 -- L_152973139/LConn1
  T_152973139_220000;110000_Station_Rheinau/RConn2 -- L_152973139/LConn2
  T_152973139_220000;110000_Station_Rheinau/RConn3 -- L_152973139/LConn3
  T_25557397_380000;220000;110000_380_kV_Umspannwerk_Großgartach/RConn4 -- L_25557397/LConn1
  T_25557397_380000;220000;110000_380_kV_Umspannwerk_Großgartach/RConn5 -- L_25557397/LConn2
  T_25557397_380000;220000;110000_380_kV_Umspannwerk_Großgartach/RConn6 -- L_25557397/LConn3
  T_166604822_380000_Markersbach/RConn1 -- L_166604822/LConn1
  T_166604822_380000_Markersbach/RConn2 -- L_166604822/LConn2
  T_166604822_380000_Markersbach/RConn3 -- L_166604822/LConn3
  T_23117075_380000;220000;110000_Umspannwerk_Röhrsdorf/RConn4 -- L_23117075/LConn1
  T_23117075_380000;220000;110000_Umspannwerk_Röhrsdorf/RConn5 -- L_23117075/LConn2
  T_23117075_380000;220000;110000_Umspannwerk_Röhrsdorf/RConn6 -- L_23117075/LConn3
  T_36183042_380000;110000_Umspannwerk_Zwönitz/RConn1 -- L_36183042/LConn1
  T_36183042_380000;110000_Umspannwerk_Zwönitz/RConn2 -- L_36183042/LConn2
  T_36183042_380000;110000_Umspannwerk_Zwönitz/RConn3 -- L_36183042/LConn3
  T_113047581_380000;220000;110000_Sottrum/RConn4 -- L_113047581/LConn1
  T_113047581_380000;220000;110000_Sottrum/RConn5 -- L_113047581/LConn2
  T_113047581_380000;220000;110000_Sottrum/RConn6 -- L_113047581/LConn3
  T_28812249_220000;110000_Wechold/RConn1 -- L_28812249/LConn1
  T_28812249_220000;110000_Wechold/RConn2 -- L_28812249/LConn2
  T_28812249_220000;110000_Wechold/RConn3 -- L_28812249/LConn3
  T_24502420_380000;220000;110000_Dollern/RConn4 -- L_24502420/LConn1
  T_24502420_380000;220000;110000_Dollern/RConn5 -- L_24502420/LConn2
  T_24502420_380000;220000;110000_Dollern/RConn6 -- L_24502420/LConn3
  T_29344008_220000;110000_Stade/RConn1 -- L_29344008/LConn1
  T_29344008_220000;110000_Stade/RConn2 -- L_29344008/LConn2
  T_29344008_220000;110000_Stade/RConn3 -- L_29344008/LConn3
  T_33017336_220000_Abbenfleth/RConn1 -- L_33017336/LConn1
  T_33017336_220000_Abbenfleth/RConn2 -- L_33017336/LConn2
  T_33017336_220000_Abbenfleth/RConn3 -- L_33017336/LConn3
  T_229565743_220000;110000_Umspannwerk_Blockland/RConn1 -- L_229565743/LConn1
  T_229565743_220000;110000_Umspannwerk_Blockland/RConn2 -- L_229565743/LConn2
  T_229565743_220000;110000_Umspannwerk_Blockland/RConn3 -- L_229565743/LConn3
  T_77038371_380000;110000_Umspannwerk_Bidingen_Nr__697_S/RConn1 -- L_77038371/LConn1
  T_77038371_380000;110000_Umspannwerk_Bidingen_Nr__697_S/RConn2 -- L_77038371/LConn2
  T_77038371_380000;110000_Umspannwerk_Bidingen_Nr__697_S/RConn3 -- L_77038371/LConn3
  T_25487161_220000;110000_Umspannwerk_Memmingen/RConn1 -- L_25487161/LConn1
  T_25487161_220000;110000_Umspannwerk_Memmingen/RConn2 -- L_25487161/LConn2
  T_25487161_220000;110000_Umspannwerk_Memmingen/RConn3 -- L_25487161/LConn3
  T_31019937_380000;220000;110000_Vöhringen_LEW/RConn4 -- L_31019937/LConn1
  T_31019937_380000;220000;110000_Vöhringen_LEW/RConn5 -- L_31019937/LConn2
  T_31019937_380000;220000;110000_Vöhringen_LEW/RConn6 -- L_31019937/LConn3
  T_85523877_380000_Vöhringen_Amprion/RConn1 -- L_85523877/LConn1
  T_85523877_380000_Vöhringen_Amprion/RConn2 -- L_85523877/LConn2
  T_85523877_380000_Vöhringen_Amprion/RConn3 -- L_85523877/LConn3
  T_27200252_220000;110000_Umspannstation_Irsingen/RConn1 -- L_27200252/LConn1
  T_27200252_220000;110000_Umspannstation_Irsingen/RConn2 -- L_27200252/LConn2
  T_27200252_220000;110000_Umspannstation_Irsingen/RConn3 -- L_27200252/LConn3
  T_30613895_380000;220000;110000_Umspannwerk_Oberottmarshausen/RConn4 -- L_30613895/LConn1
  T_30613895_380000;220000;110000_Umspannwerk_Oberottmarshausen/RConn5 -- L_30613895/LConn2
  T_30613895_380000;220000;110000_Umspannwerk_Oberottmarshausen/RConn6 -- L_30613895/LConn3
  T_34414970_220000;110000_Umspannwerk_Rauhenzell/RConn1 -- L_34414970/LConn1
  T_34414970_220000;110000_Umspannwerk_Rauhenzell/RConn2 -- L_34414970/LConn2
  T_34414970_220000;110000_Umspannwerk_Rauhenzell/RConn3 -- L_34414970/LConn3
  T_46766896_220000_Schaltwerk_Kempten/RConn1 -- L_46766896/LConn1
  T_46766896_220000_Schaltwerk_Kempten/RConn2 -- L_46766896/LConn2
  T_46766896_220000_Schaltwerk_Kempten/RConn3 -- L_46766896/LConn3
  T_147521567_220000;110000_Umspannanlage_Pfungstadt/RConn1 -- L_147521567/LConn1
  T_147521567_220000;110000_Umspannanlage_Pfungstadt/RConn2 -- L_147521567/LConn2
  T_147521567_220000;110000_Umspannanlage_Pfungstadt/RConn3 -- L_147521567/LConn3
  T_152022992_220000;110000_Niederhausen/RConn1 -- L_152022992/LConn1
  T_152022992_220000;110000_Niederhausen/RConn2 -- L_152022992/LConn2
  T_152022992_220000;110000_Niederhausen/RConn3 -- L_152022992/LConn3
  T_177829920_380000;150000;110000_Diele/RConn1 -- L_177829920/LConn1
  T_177829920_380000;150000;110000_Diele/RConn2 -- L_177829920/LConn2
  T_177829920_380000;150000;110000_Diele/RConn3 -- L_177829920/LConn3
  T_23837631_380000;220000;110000_Conneforde/RConn4 -- L_23837631/LConn1
  T_23837631_380000;220000;110000_Conneforde/RConn5 -- L_23837631/LConn2
  T_23837631_380000;220000;110000_Conneforde/RConn6 -- L_23837631/LConn3
  T_32042992_380000_Umspannwerk_Rhede/RConn1 -- L_32042992/LConn1
  T_32042992_380000_Umspannwerk_Rhede/RConn2 -- L_32042992/LConn2
  T_32042992_380000_Umspannwerk_Rhede/RConn3 -- L_32042992/LConn3
  T_25306752_380000;220000;110000_Umspannwerk_Herbertingen/RConn4 -- L_25306752/LConn1
  T_25306752_380000;220000;110000_Umspannwerk_Herbertingen/RConn5 -- L_25306752/LConn2
  T_25306752_380000;220000;110000_Umspannwerk_Herbertingen/RConn6 -- L_25306752/LConn3
  T_25802269_380000;220000;110000_Umspannstation_Hoheneck_Amprion/RConn4 -- L_25802269/LConn1
  T_25802269_380000;220000;110000_Umspannstation_Hoheneck_Amprion/RConn5 -- L_25802269/LConn2
  T_25802269_380000;220000;110000_Umspannstation_Hoheneck_Amprion/RConn6 -- L_25802269/LConn3
  T_97825259_220000;110000_Marbach/RConn1 -- L_97825259/LConn1
  T_97825259_220000;110000_Marbach/RConn2 -- L_97825259/LConn2
  T_97825259_220000;110000_Marbach/RConn3 -- L_97825259/LConn3
  T_32205824_220000;110000_Umspannwerk_Winnenden/RConn1 -- L_32205824/LConn1
  T_32205824_220000;110000_Umspannwerk_Winnenden/RConn2 -- L_32205824/LConn2
  T_32205824_220000;110000_Umspannwerk_Winnenden/RConn3 -- L_32205824/LConn3
  T_26260052_380000;220000;110000_EnBW_Umspannwerk_Wendlingen/RConn4 -- L_26260052/LConn1
  T_26260052_380000;220000;110000_EnBW_Umspannwerk_Wendlingen/RConn5 -- L_26260052/LConn2
  T_26260052_380000;220000;110000_EnBW_Umspannwerk_Wendlingen/RConn6 -- L_26260052/LConn3
  T_115808262__/RConn1 -- L_115808262/LConn1
  T_115808262__/RConn2 -- L_115808262/LConn2
  T_115808262__/RConn3 -- L_115808262/LConn3
  T_26593929_380000;110000_Station_Oberzier/RConn1 -- L_26593929/LConn1
  T_26593929_380000;110000_Station_Oberzier/RConn2 -- L_26593929/LConn2
  T_26593929_380000;110000_Station_Oberzier/RConn3 -- L_26593929/LConn3
  T_24268944_380000;110000_Station_Verlautenheide/RConn1 -- L_24268944/LConn1
  T_24268944_380000;110000_Station_Verlautenheide/RConn2 -- L_24268944/LConn2
  T_24268944_380000;110000_Station_Verlautenheide/RConn3 -- L_24268944/LConn3
  T_25426571_380000;110000_Umspannwerk_Weisweiler/RConn1 -- L_25426571/LConn1
  T_25426571_380000;110000_Umspannwerk_Weisweiler/RConn2 -- L_25426571/LConn2
  T_25426571_380000;110000_Umspannwerk_Weisweiler/RConn3 -- L_25426571/LConn3
  T_31105067_380000;110000_Umspannwerk_Niederstotzingen/RConn1 -- L_31105067/LConn1
  T_31105067_380000;110000_Umspannwerk_Niederstotzingen/RConn2 -- L_31105067/LConn2
  T_31105067_380000;110000_Umspannwerk_Niederstotzingen/RConn3 -- L_31105067/LConn3
  T_38325076_380000;110000_Umspannwerk_Rotensohl/RConn1 -- L_38325076/LConn1
  T_38325076_380000;110000_Umspannwerk_Rotensohl/RConn2 -- L_38325076/LConn2
  T_38325076_380000;110000_Umspannwerk_Rotensohl/RConn3 -- L_38325076/LConn3
  T_42050342_380000;220000;110000_Umspannwerk_Goldshöfe/RConn4 -- L_42050342/LConn1
  T_42050342_380000;220000;110000_Umspannwerk_Goldshöfe/RConn5 -- L_42050342/LConn2
  T_42050342_380000;220000;110000_Umspannwerk_Goldshöfe/RConn6 -- L_42050342/LConn3
  T_41389594_380000;220000;110000_Umspannwerk_Dellmensingen/RConn4 -- L_41389594/LConn1
  T_41389594_380000;220000;110000_Umspannwerk_Dellmensingen/RConn5 -- L_41389594/LConn2
  T_41389594_380000;220000;110000_Umspannwerk_Dellmensingen/RConn6 -- L_41389594/LConn3
  T_130794504_220000;110000_Lübeck/RConn1 -- L_130794504/LConn1
  T_130794504_220000;110000_Lübeck/RConn2 -- L_130794504/LConn2
  T_130794504_220000;110000_Lübeck/RConn3 -- L_130794504/LConn3
  T_28008024_220000;110000;30000_Hamburg_Nord/RConn1 -- L_28008024/LConn1
  T_28008024_220000;110000;30000_Hamburg_Nord/RConn2 -- L_28008024/LConn2
  T_28008024_220000;110000;30000_Hamburg_Nord/RConn3 -- L_28008024/LConn3
  T_87767090__Station_Mettmann/RConn1 -- L_87767090/LConn1
  T_87767090__Station_Mettmann/RConn2 -- L_87767090/LConn2
  T_87767090__Station_Mettmann/RConn3 -- L_87767090/LConn3
  T_87767098_220000_Station_Mettmann/RConn1 -- L_87767098/LConn1
  T_87767098_220000_Station_Mettmann/RConn2 -- L_87767098/LConn2
  T_87767098_220000_Station_Mettmann/RConn3 -- L_87767098/LConn3
  T_32063539_380000_Bentwisch_HGÜ/RConn1 -- L_32063539/LConn1
  T_32063539_380000_Bentwisch_HGÜ/RConn2 -- L_32063539/LConn2
  T_32063539_380000_Bentwisch_HGÜ/RConn3 -- L_32063539/LConn3
  T_33745279__/RConn1 -- L_33745279/LConn1
  T_33745279__/RConn2 -- L_33745279/LConn2
  T_33745279__/RConn3 -- L_33745279/LConn3
  T_24758329_380000;110000_Umspannwerk_Eltmann/RConn1 -- L_24758329/LConn1
  T_24758329_380000;110000_Umspannwerk_Eltmann/RConn2 -- L_24758329/LConn2
  T_24758329_380000;110000_Umspannwerk_Eltmann/RConn3 -- L_24758329/LConn3
  T_108797675_380000_Grafenrheinfeld/RConn1 -- L_108797675/LConn1
  T_108797675_380000_Grafenrheinfeld/RConn2 -- L_108797675/LConn2
  T_108797675_380000_Grafenrheinfeld/RConn3 -- L_108797675/LConn3
  T_24715381_380000;220000;110000_Umspannwerk_Bergrheinfeld/RConn4 -- L_24715381/LConn1
  T_24715381_380000;220000;110000_Umspannwerk_Bergrheinfeld/RConn5 -- L_24715381/LConn2
  T_24715381_380000;220000;110000_Umspannwerk_Bergrheinfeld/RConn6 -- L_24715381/LConn3
  T_24757393__Umspannwerk_Würgau/RConn1 -- L_24757393/LConn1
  T_24757393__Umspannwerk_Würgau/RConn2 -- L_24757393/LConn2
  T_24757393__Umspannwerk_Würgau/RConn3 -- L_24757393/LConn3
  T_24705761_380000;220000;110000_Umspannwerk_Raitersaich/RConn4 -- L_24705761/LConn1
  T_24705761_380000;220000;110000_Umspannwerk_Raitersaich/RConn5 -- L_24705761/LConn2
  T_24705761_380000;220000;110000_Umspannwerk_Raitersaich/RConn6 -- L_24705761/LConn3
  T_28613721_380000;110000_Kriegenbrunn/RConn1 -- L_28613721/LConn1
  T_28613721_380000;110000_Kriegenbrunn/RConn2 -- L_28613721/LConn2
  T_28613721_380000;110000_Kriegenbrunn/RConn3 -- L_28613721/LConn3
  T_24757392_380000;110000_Umspannwerk_Redwitz/RConn1 -- L_24757392/LConn1
  T_24757392_380000;110000_Umspannwerk_Redwitz/RConn2 -- L_24757392/LConn2
  T_24757392_380000;110000_Umspannwerk_Redwitz/RConn3 -- L_24757392/LConn3
  T_24757833_380000_Umspannwerk_Oberhaid/RConn1 -- L_24757833/LConn1
  T_24757833_380000_Umspannwerk_Oberhaid/RConn2 -- L_24757833/LConn2
  T_24757833_380000_Umspannwerk_Oberhaid/RConn3 -- L_24757833/LConn3
  T_23192640_220000;110000_Station_Reisholz/RConn1 -- L_23192640/LConn1
  T_23192640_220000;110000_Station_Reisholz/RConn2 -- L_23192640/LConn2
  T_23192640_220000;110000_Station_Reisholz/RConn3 -- L_23192640/LConn3
  T_-1897787__Station_Sankt_Peter/RConn1 -- L_-1897787/LConn1
  T_-1897787__Station_Sankt_Peter/RConn2 -- L_-1897787/LConn2
  T_-1897787__Station_Sankt_Peter/RConn3 -- L_-1897787/LConn3
  T_23140544_220000;110000_Station_Eller/RConn1 -- L_23140544/LConn1
  T_23140544_220000;110000_Station_Eller/RConn2 -- L_23140544/LConn2
  T_23140544_220000;110000_Station_Eller/RConn3 -- L_23140544/LConn3
  T_22761839_380000;220000;110000_Station_Opladen/RConn4 -- L_22761839/LConn1
  T_22761839_380000;220000;110000_Station_Opladen/RConn5 -- L_22761839/LConn2
  T_22761839_380000;220000;110000_Station_Opladen/RConn6 -- L_22761839/LConn3
  T_35954395_380000;110000_Umspannwerk_Trossingen/RConn1 -- L_35954395/LConn1
  T_35954395_380000;110000_Umspannwerk_Trossingen/RConn2 -- L_35954395/LConn2
  T_35954395_380000;110000_Umspannwerk_Trossingen/RConn3 -- L_35954395/LConn3
  T_42736239_380000_EnBW_Umspannwerk_Engstlatt/RConn1 -- L_42736239/LConn1
  T_42736239_380000_EnBW_Umspannwerk_Engstlatt/RConn2 -- L_42736239/LConn2
  T_42736239_380000_EnBW_Umspannwerk_Engstlatt/RConn3 -- L_42736239/LConn3
  T_42049947_380000;110000_Umspannwerk_Villingen/RConn1 -- L_42049947/LConn1
  T_42049947_380000;110000_Umspannwerk_Villingen/RConn2 -- L_42049947/LConn2
  T_42049947_380000;110000_Umspannwerk_Villingen/RConn3 -- L_42049947/LConn3
  T_88901626_380000;110000_Schwörstadt/RConn1 -- L_88901626/LConn1
  T_88901626_380000;110000_Schwörstadt/RConn2 -- L_88901626/LConn2
  T_88901626_380000;110000_Schwörstadt/RConn3 -- L_88901626/LConn3
  T_242756113_380000;220000;110000_380_kV_Umspannwerk_Eichstetten/RConn4 -- L_242756113/LConn1
  T_242756113_380000;220000;110000_380_kV_Umspannwerk_Eichstetten/RConn5 -- L_242756113/LConn2
  T_242756113_380000;220000;110000_380_kV_Umspannwerk_Eichstetten/RConn6 -- L_242756113/LConn3
  T_152261133_380000;220000;110000_Karlsruhe_Daxlanden/RConn4 -- L_152261133/LConn1
  T_152261133_380000;220000;110000_Karlsruhe_Daxlanden/RConn5 -- L_152261133/LConn2
  T_152261133_380000;220000;110000_Karlsruhe_Daxlanden/RConn6 -- L_152261133/LConn3
  T_129790129__/RConn1 -- L_129790129/LConn1
  T_129790129__/RConn2 -- L_129790129/LConn2
  T_129790129__/RConn3 -- L_129790129/LConn3
  T_31367940_380000;220000;110000_Tiengen/RConn4 -- L_31367940/LConn1
  T_31367940_380000;220000;110000_Tiengen/RConn5 -- L_31367940/LConn2
  T_31367940_380000;220000;110000_Tiengen/RConn6 -- L_31367940/LConn3
  T_202865176_220000_/RConn1 -- L_202865176/LConn1
  T_202865176_220000_/RConn2 -- L_202865176/LConn2
  T_202865176_220000_/RConn3 -- L_202865176/LConn3
  T_202865177_380000_Kabelanfang_PSP_Wehr/RConn1 -- L_202865177/LConn1
  T_202865177_380000_Kabelanfang_PSP_Wehr/RConn2 -- L_202865177/LConn2
  T_202865177_380000_Kabelanfang_PSP_Wehr/RConn3 -- L_202865177/LConn3
  T_32151621_220000;110000_220_kV_Umspannwerk_Kuppenheim/RConn1 -- L_32151621/LConn1
  T_32151621_220000;110000_220_kV_Umspannwerk_Kuppenheim/RConn2 -- L_32151621/LConn2
  T_32151621_220000;110000_220_kV_Umspannwerk_Kuppenheim/RConn3 -- L_32151621/LConn3
  T_39011884_220000;110000_Bühl/RConn1 -- L_39011884/LConn1
  T_39011884_220000;110000_Bühl/RConn2 -- L_39011884/LConn2
  T_39011884_220000;110000_Bühl/RConn3 -- L_39011884/LConn3
  T_146962222_220000;110000_Umspannwerk_Weier/RConn1 -- L_146962222/LConn1
  T_146962222_220000;110000_Umspannwerk_Weier/RConn2 -- L_146962222/LConn2
  T_146962222_220000;110000_Umspannwerk_Weier/RConn3 -- L_146962222/LConn3
  T_89184327__/RConn1 -- L_89184327/LConn1
  T_89184327__/RConn2 -- L_89184327/LConn2
  T_89184327__/RConn3 -- L_89184327/LConn3
  T_137602559_380000;220000;110000_Irsching/RConn4 -- L_137602559/LConn1
  T_137602559_380000;220000;110000_Irsching/RConn5 -- L_137602559/LConn2
  T_137602559_380000;220000;110000_Irsching/RConn6 -- L_137602559/LConn3
  T_18629425_380000;220000;110000_Umspannwerk_Oberbachern/RConn4 -- L_18629425/LConn1
  T_18629425_380000;220000;110000_Umspannwerk_Oberbachern/RConn5 -- L_18629425/LConn2
  T_18629425_380000;220000;110000_Umspannwerk_Oberbachern/RConn6 -- L_18629425/LConn3
  T_24158385_220000;110000_Umspannwerk_Neufinsing/RConn1 -- L_24158385/LConn1
  T_24158385_220000;110000_Umspannwerk_Neufinsing/RConn2 -- L_24158385/LConn2
  T_24158385_220000;110000_Umspannwerk_Neufinsing/RConn3 -- L_24158385/LConn3
  T_5404079_380000;110000_Föhring/RConn1 -- L_5404079/LConn1
  T_5404079_380000;110000_Föhring/RConn2 -- L_5404079/LConn2
  T_5404079_380000;110000_Föhring/RConn3 -- L_5404079/LConn3
  T_29374542_220000;110000_Station_Gremberghoven/RConn1 -- L_29374542/LConn1
  T_29374542_220000;110000_Station_Gremberghoven/RConn2 -- L_29374542/LConn2
  T_29374542_220000;110000_Station_Gremberghoven/RConn3 -- L_29374542/LConn3
  T_27871140_220000_Station_Dünnwald/RConn1 -- L_27871140/LConn1
  T_27871140_220000_Station_Dünnwald/RConn2 -- L_27871140/LConn2
  T_27871140_220000_Station_Dünnwald/RConn3 -- L_27871140/LConn3
  T_22767509_220000;110000_Station_Siegburg/RConn1 -- L_22767509/LConn1
  T_22767509_220000;110000_Station_Siegburg/RConn2 -- L_22767509/LConn2
  T_22767509_220000;110000_Station_Siegburg/RConn3 -- L_22767509/LConn3
  T_22796434_220000;110000_Station_Stockem/RConn1 -- L_22796434/LConn1
  T_22796434_220000;110000_Station_Stockem/RConn2 -- L_22796434/LConn2
  T_22796434_220000;110000_Station_Stockem/RConn3 -- L_22796434/LConn3
  T_29472852_220000;110000_Station_Ibbenbüren/RConn1 -- L_29472852/LConn1
  T_29472852_220000;110000_Station_Ibbenbüren/RConn2 -- L_29472852/LConn2
  T_29472852_220000;110000_Station_Ibbenbüren/RConn3 -- L_29472852/LConn3
  T_114319248_380000;220000;110000_Station_Westerkappeln/RConn4 -- L_114319248/LConn1
  T_114319248_380000;220000;110000_Station_Westerkappeln/RConn5 -- L_114319248/LConn2
  T_114319248_380000;220000;110000_Station_Westerkappeln/RConn6 -- L_114319248/LConn3
  T_37764852_220000;110000_Station_Lüstringen/RConn1 -- L_37764852/LConn1
  T_37764852_220000;110000_Station_Lüstringen/RConn2 -- L_37764852/LConn2
  T_37764852_220000;110000_Station_Lüstringen/RConn3 -- L_37764852/LConn3
  T_42861703_220000_Amelsbüren/RConn1 -- L_42861703/LConn1
  T_42861703_220000_Amelsbüren/RConn2 -- L_42861703/LConn2
  T_42861703_220000_Amelsbüren/RConn3 -- L_42861703/LConn3
  T_61918154_380000;220000;110000_Hanekenfähr/RConn4 -- L_61918154/LConn1
  T_61918154_380000;220000;110000_Hanekenfähr/RConn5 -- L_61918154/LConn2
  T_61918154_380000;220000;110000_Hanekenfähr/RConn6 -- L_61918154/LConn3
  T_29077623_380000;220000;110000_Station_Kusenhorst/RConn4 -- L_29077623/LConn1
  T_29077623_380000;220000;110000_Station_Kusenhorst/RConn5 -- L_29077623/LConn2
  T_29077623_380000;220000;110000_Station_Kusenhorst/RConn6 -- L_29077623/LConn3
  T_202164315_380000_KW_Heyden/RConn1 -- L_202164315/LConn1
  T_202164315_380000_KW_Heyden/RConn2 -- L_202164315/LConn2
  T_202164315_380000_KW_Heyden/RConn3 -- L_202164315/LConn3
  T_24604789_380000_Schaltanlage_Ovenstädt/RConn1 -- L_24604789/LConn1
  T_24604789_380000_Schaltanlage_Ovenstädt/RConn2 -- L_24604789/LConn2
  T_24604789_380000_Schaltanlage_Ovenstädt/RConn3 -- L_24604789/LConn3
  T_136034396_380000;320000;250000_Konverterstation_Büttel/RConn1 -- L_136034396/LConn1
  T_136034396_380000;320000;250000_Konverterstation_Büttel/RConn2 -- L_136034396/LConn2
  T_136034396_380000;320000;250000_Konverterstation_Büttel/RConn3 -- L_136034396/LConn3
  T_28502915_380000_Umspannwerk_Wilster/RConn1 -- L_28502915/LConn1
  T_28502915_380000_Umspannwerk_Wilster/RConn2 -- L_28502915/LConn2
  T_28502915_380000_Umspannwerk_Wilster/RConn3 -- L_28502915/LConn3
  T_30622610_380000;220000;110000_Umspannwerk_Kernkraftwerk_Brunsbüttel/RConn4 -- L_30622610/LConn1
  T_30622610_380000;220000;110000_Umspannwerk_Kernkraftwerk_Brunsbüttel/RConn5 -- L_30622610/LConn2
  T_30622610_380000;220000;110000_Umspannwerk_Kernkraftwerk_Brunsbüttel/RConn6 -- L_30622610/LConn3
  T_93341407_380000;220000;110000_Umspannwerk_Mechlenreuth/RConn4 -- L_93341407/LConn1
  T_93341407_380000;220000;110000_Umspannwerk_Mechlenreuth/RConn5 -- L_93341407/LConn2
  T_93341407_380000;220000;110000_Umspannwerk_Mechlenreuth/RConn6 -- L_93341407/LConn3
  T_29084374_380000;110000_Umspannwerk_Etzenricht/RConn1 -- L_29084374/LConn1
  T_29084374_380000;110000_Umspannwerk_Etzenricht/RConn2 -- L_29084374/LConn2
  T_29084374_380000;110000_Umspannwerk_Etzenricht/RConn3 -- L_29084374/LConn3
  T_28956649_380000;220000;110000_Schwandorf/RConn4 -- L_28956649/LConn1
  T_28956649_380000;220000;110000_Schwandorf/RConn5 -- L_28956649/LConn2
  T_28956649_380000;220000;110000_Schwandorf/RConn6 -- L_28956649/LConn3
  T_91080806_220000;110000_Umspannwerk_Pirach/RConn1 -- L_91080806/LConn1
  T_91080806_220000;110000_Umspannwerk_Pirach/RConn2 -- L_91080806/LConn2
  T_91080806_220000;110000_Umspannwerk_Pirach/RConn3 -- L_91080806/LConn3
  T_173590639_220000;110000_Niederwiesa/RConn1 -- L_173590639/LConn1
  T_173590639_220000;110000_Niederwiesa/RConn2 -- L_173590639/LConn2
  T_173590639_220000;110000_Niederwiesa/RConn3 -- L_173590639/LConn3
  T_24479857_220000;110000_Station_Gellep/RConn1 -- L_24479857/LConn1
  T_24479857_220000;110000_Station_Gellep/RConn2 -- L_24479857/LConn2
  T_24479857_220000;110000_Station_Gellep/RConn3 -- L_24479857/LConn3
  T_24799890_220000;110000_Station_Osterath/RConn1 -- L_24799890/LConn1
  T_24799890_220000;110000_Station_Osterath/RConn2 -- L_24799890/LConn2
  T_24799890_220000;110000_Station_Osterath/RConn3 -- L_24799890/LConn3
  T_91854336_220000;110000_Station_Mündelheim/RConn1 -- L_91854336/LConn1
  T_91854336_220000;110000_Station_Mündelheim/RConn2 -- L_91854336/LConn2
  T_91854336_220000;110000_Station_Mündelheim/RConn3 -- L_91854336/LConn3
  T_92024105_220000_Station_Rheinhausen/RConn1 -- L_92024105/LConn1
  T_92024105_220000_Station_Rheinhausen/RConn2 -- L_92024105/LConn2
  T_92024105_220000_Station_Rheinhausen/RConn3 -- L_92024105/LConn3
  T_25043127_220000;110000_Station_Selbeck/RConn1 -- L_25043127/LConn1
  T_25043127_220000;110000_Station_Selbeck/RConn2 -- L_25043127/LConn2
  T_25043127_220000;110000_Station_Selbeck/RConn3 -- L_25043127/LConn3
  T_276236628_220000;110000_Schweinfurt/RConn1 -- L_276236628/LConn1
  T_276236628_220000;110000_Schweinfurt/RConn2 -- L_276236628/LConn2
  T_276236628_220000;110000_Schweinfurt/RConn3 -- L_276236628/LConn3
  T_38584673_220000_Station_Bellendorf/RConn1 -- L_38584673/LConn1
  T_38584673_220000_Station_Bellendorf/RConn2 -- L_38584673/LConn2
  T_38584673_220000_Station_Bellendorf/RConn3 -- L_38584673/LConn3
  T_22944791_220000;110000_Station_Bergmannsglück/RConn1 -- L_22944791/LConn1
  T_22944791_220000;110000_Station_Bergmannsglück/RConn2 -- L_22944791/LConn2
  T_22944791_220000;110000_Station_Bergmannsglück/RConn3 -- L_22944791/LConn3
  T_68549340_220000;110000_Station_Bochum/RConn1 -- L_68549340/LConn1
  T_68549340_220000;110000_Station_Bochum/RConn2 -- L_68549340/LConn2
  T_68549340_220000;110000_Station_Bochum/RConn3 -- L_68549340/LConn3
  T_29282738_220000;110000_Herne/RConn1 -- L_29282738/LConn1
  T_29282738_220000;110000_Herne/RConn2 -- L_29282738/LConn2
  T_29282738_220000;110000_Herne/RConn3 -- L_29282738/LConn3
  T_32472806_380000_Station_Mengede/RConn1 -- L_32472806/LConn1
  T_32472806_380000_Station_Mengede/RConn2 -- L_32472806/LConn2
  T_32472806_380000_Station_Mengede/RConn3 -- L_32472806/LConn3
  T_23067006_380000;110000_Station_Hüllen/RConn1 -- L_23067006/LConn1
  T_23067006_380000;110000_Station_Hüllen/RConn2 -- L_23067006/LConn2
  T_23067006_380000;110000_Station_Hüllen/RConn3 -- L_23067006/LConn3
  T_63114179_380000;220000;110000_Station_Hattingen/RConn4 -- L_63114179/LConn1
  T_63114179_380000;220000;110000_Station_Hattingen/RConn5 -- L_63114179/LConn2
  T_63114179_380000;220000;110000_Station_Hattingen/RConn6 -- L_63114179/LConn3
  T_29471404_380000;220000;110000_Station_Gronau/RConn1 -- L_29471404/LConn1
  T_29471404_380000;220000;110000_Station_Gronau/RConn2 -- L_29471404/LConn2
  T_29471404_380000;220000;110000_Station_Gronau/RConn3 -- L_29471404/LConn3
  T_26383042_380000;220000;110000;10000_Umspannwerk_Blankenhagen/RConn4 -- L_26383042/LConn1
  T_26383042_380000;220000;110000;10000_Umspannwerk_Blankenhagen/RConn5 -- L_26383042/LConn2
  T_26383042_380000;220000;110000;10000_Umspannwerk_Blankenhagen/RConn6 -- L_26383042/LConn3
  T_42560068_380000;110000_Station_Enniger/RConn1 -- L_42560068/LConn1
  T_42560068_380000;110000_Station_Enniger/RConn2 -- L_42560068/LConn2
  T_42560068_380000;110000_Station_Enniger/RConn3 -- L_42560068/LConn3
  T_42488850_380000_Station_Uentrop/RConn1 -- L_42488850/LConn1
  T_42488850_380000_Station_Uentrop/RConn2 -- L_42488850/LConn2
  T_42488850_380000_Station_Uentrop/RConn3 -- L_42488850/LConn3
  T_25506770_380000;110000_Station_Roxel/RConn1 -- L_25506770/LConn1
  T_25506770_380000;110000_Station_Roxel/RConn2 -- L_25506770/LConn2
  T_25506770_380000;110000_Station_Roxel/RConn3 -- L_25506770/LConn3
  T_206289192_380000;110000_Meppen/RConn1 -- L_206289192/LConn1
  T_206289192_380000;110000_Meppen/RConn2 -- L_206289192/LConn2
  T_206289192_380000;110000_Meppen/RConn3 -- L_206289192/LConn3
  T_142487746_380000;320000_Dörpen_West/RConn1 -- L_142487746/LConn1
  T_142487746_380000;320000_Dörpen_West/RConn2 -- L_142487746/LConn2
  T_142487746_380000;320000_Dörpen_West/RConn3 -- L_142487746/LConn3
  T_49299111_380000;110000_Niederlangen/RConn1 -- L_49299111/LConn1
  T_49299111_380000;110000_Niederlangen/RConn2 -- L_49299111/LConn2
  T_49299111_380000;110000_Niederlangen/RConn3 -- L_49299111/LConn3
  T_33411203_380000;220000;110000_Wehrendorf/RConn4 -- L_33411203/LConn1
  T_33411203_380000;220000;110000_Wehrendorf/RConn5 -- L_33411203/LConn2
  T_33411203_380000;220000;110000_Wehrendorf/RConn6 -- L_33411203/LConn3
  T_39690368_220000;110000_Güstrow/RConn1 -- L_39690368/LConn1
  T_39690368_220000;110000_Güstrow/RConn2 -- L_39690368/LConn2
  T_39690368_220000;110000_Güstrow/RConn3 -- L_39690368/LConn3
  T_32904794_220000;110000_Station_Sankt_Hülfe/RConn1 -- L_32904794/LConn1
  T_32904794_220000;110000_Station_Sankt_Hülfe/RConn2 -- L_32904794/LConn2
  T_32904794_220000;110000_Station_Sankt_Hülfe/RConn3 -- L_32904794/LConn3
  T_22720647_380000;220000;110000_Umspannwerk_Hamburg_Nord/RConn4 -- L_22720647/LConn1
  T_22720647_380000;220000;110000_Umspannwerk_Hamburg_Nord/RConn5 -- L_22720647/LConn2
  T_22720647_380000;220000;110000_Umspannwerk_Hamburg_Nord/RConn6 -- L_22720647/LConn3
  T_23583867_380000;110000_Umspannwerk_Hamburg_Ost/RConn1 -- L_23583867/LConn1
  T_23583867_380000;110000_Umspannwerk_Hamburg_Ost/RConn2 -- L_23583867/LConn2
  T_23583867_380000;110000_Umspannwerk_Hamburg_Ost/RConn3 -- L_23583867/LConn3
  T_42488855_380000;110000_Station_Lippborg/RConn1 -- L_42488855/LConn1
  T_42488855_380000;110000_Station_Lippborg/RConn2 -- L_42488855/LConn2
  T_42488855_380000;110000_Station_Lippborg/RConn3 -- L_42488855/LConn3
  T_112695048_380000_Geithe/RConn1 -- L_112695048/LConn1
  T_112695048_380000_Geithe/RConn2 -- L_112695048/LConn2
  T_112695048_380000_Geithe/RConn3 -- L_112695048/LConn3
  T_42809973_380000;110000_Station_Unna/RConn1 -- L_42809973/LConn1
  T_42809973_380000;110000_Station_Unna/RConn2 -- L_42809973/LConn2
  T_42809973_380000;110000_Station_Unna/RConn3 -- L_42809973/LConn3
  T_35763480_380000_Witten/RConn1 -- L_35763480/LConn1
  T_35763480_380000_Witten/RConn2 -- L_35763480/LConn2
  T_35763480_380000_Witten/RConn3 -- L_35763480/LConn3
  T_22964137_380000;220000;110000_Station_Kruckel/RConn1 -- L_22964137/LConn1
  T_22964137_380000;220000;110000_Station_Kruckel/RConn2 -- L_22964137/LConn2
  T_22964137_380000;220000;110000_Station_Kruckel/RConn3 -- L_22964137/LConn3
  T_59707532_380000;110000_Umspannwerk_Perleberg/RConn1 -- L_59707532/LConn1
  T_59707532_380000;110000_Umspannwerk_Perleberg/RConn2 -- L_59707532/LConn2
  T_59707532_380000;110000_Umspannwerk_Perleberg/RConn3 -- L_59707532/LConn3
  T_33169401_380000;110000_Stendal_West/RConn1 -- L_33169401/LConn1
  T_33169401_380000;110000_Stendal_West/RConn2 -- L_33169401/LConn2
  T_33169401_380000;110000_Stendal_West/RConn3 -- L_33169401/LConn3
  T_369680693_380000;110000_Siedenbrünzow/RConn1 -- L_369680693/LConn1
  T_369680693_380000;110000_Siedenbrünzow/RConn2 -- L_369680693/LConn2
  T_369680693_380000;110000_Siedenbrünzow/RConn3 -- L_369680693/LConn3
  T_66764943_220000;110000_Station_Wengerohr/RConn1 -- L_66764943/LConn1
  T_66764943_220000;110000_Station_Wengerohr/RConn2 -- L_66764943/LConn2
  T_66764943_220000;110000_Station_Wengerohr/RConn3 -- L_66764943/LConn3
  T_145680894_220000_Station_Trier/RConn1 -- L_145680894/LConn1
  T_145680894_220000_Station_Trier/RConn2 -- L_145680894/LConn2
  T_145680894_220000_Station_Trier/RConn3 -- L_145680894/LConn3
  T_151967291_220000;110000_Station_Quint/RConn1 -- L_151967291/LConn1
  T_151967291_220000;110000_Station_Quint/RConn2 -- L_151967291/LConn2
  T_151967291_220000;110000_Station_Quint/RConn3 -- L_151967291/LConn3
  T_54359256_380000;220000;110000_Umspannwerk_Uchtelfangen/RConn4 -- L_54359256/LConn1
  T_54359256_380000;220000;110000_Umspannwerk_Uchtelfangen/RConn5 -- L_54359256/LConn2
  T_54359256_380000;220000;110000_Umspannwerk_Uchtelfangen/RConn6 -- L_54359256/LConn3
  T_89352550_380000;220000;110000_Bexbach_Kraftwerk/RConn4 -- L_89352550/LConn1
  T_89352550_380000;220000;110000_Bexbach_Kraftwerk/RConn5 -- L_89352550/LConn2
  T_89352550_380000;220000;110000_Bexbach_Kraftwerk/RConn6 -- L_89352550/LConn3
  T_156402422_220000;110000_Beeden/RConn1 -- L_156402422/LConn1
  T_156402422_220000;110000_Beeden/RConn2 -- L_156402422/LConn2
  T_156402422_220000;110000_Beeden/RConn3 -- L_156402422/LConn3
  T_152107810_220000;110000_Umspannwerk_Kerzenheim/RConn1 -- L_152107810/LConn1
  T_152107810_220000;110000_Umspannwerk_Kerzenheim/RConn2 -- L_152107810/LConn2
  T_152107810_220000;110000_Umspannwerk_Kerzenheim/RConn3 -- L_152107810/LConn3
  T_276249131_220000;110000_Umspannwerk_Maximiliansau/RConn1 -- L_276249131/LConn1
  T_276249131_220000;110000_Umspannwerk_Maximiliansau/RConn2 -- L_276249131/LConn2
  T_276249131_220000;110000_Umspannwerk_Maximiliansau/RConn3 -- L_276249131/LConn3
  T_152924498_220000;110000_Netzleitstelle_Mutterstadt/RConn1 -- L_152924498/LConn1
  T_152924498_220000;110000_Netzleitstelle_Mutterstadt/RConn2 -- L_152924498/LConn2
  T_152924498_220000;110000_Netzleitstelle_Mutterstadt/RConn3 -- L_152924498/LConn3
  T_152924508_220000_BASF/RConn1 -- L_152924508/LConn1
  T_152924508_220000_BASF/RConn2 -- L_152924508/LConn2
  T_152924508_220000_BASF/RConn3 -- L_152924508/LConn3
  T_152107815_220000;110000_Otterbach/RConn1 -- L_152107815/LConn1
  T_152107815_220000;110000_Otterbach/RConn2 -- L_152107815/LConn2
  T_152107815_220000;110000_Otterbach/RConn3 -- L_152107815/LConn3
  T_151967290_380000;220000;110000_Station_Niederstedem/RConn4 -- L_151967290/LConn1
  T_151967290_380000;220000;110000_Station_Niederstedem/RConn5 -- L_151967290/LConn2
  T_151967290_380000;220000;110000_Station_Niederstedem/RConn6 -- L_151967290/LConn3
  T_395847307_380000;220000;110000_Station_Weißenthurm/RConn4 -- L_395847307/LConn1
  T_395847307_380000;220000;110000_Station_Weißenthurm/RConn5 -- L_395847307/LConn2
  T_395847307_380000;220000;110000_Station_Weißenthurm/RConn6 -- L_395847307/LConn3
  T_89215122_220000;110000_Station_Saarwellingen/RConn1 -- L_89215122/LConn1
  T_89215122_220000;110000_Station_Saarwellingen/RConn2 -- L_89215122/LConn2
  T_89215122_220000;110000_Station_Saarwellingen/RConn3 -- L_89215122/LConn3
  T_82310607_220000_Dieffeln/RConn1 -- L_82310607/LConn1
  T_82310607_220000_Dieffeln/RConn2 -- L_82310607/LConn2
  T_82310607_220000_Dieffeln/RConn3 -- L_82310607/LConn3
  T_31927411_380000;110000_Alfstedt/RConn1 -- L_31927411/LConn1
  T_31927411_380000;110000_Alfstedt/RConn2 -- L_31927411/LConn2
  T_31927411_380000;110000_Alfstedt/RConn3 -- L_31927411/LConn3
  T_11285720_380000;110000_Umspannwerk_Hamburg_Süd/RConn1 -- L_11285720/LConn1
  T_11285720_380000;110000_Umspannwerk_Hamburg_Süd/RConn2 -- L_11285720/LConn2
  T_11285720_380000;110000_Umspannwerk_Hamburg_Süd/RConn3 -- L_11285720/LConn3
  T_33816726_380000;110000_Station_Halfeshof/RConn1 -- L_33816726/LConn1
  T_33816726_380000;110000_Station_Halfeshof/RConn2 -- L_33816726/LConn2
  T_33816726_380000;110000_Station_Halfeshof/RConn3 -- L_33816726/LConn3
  T_152403632_380000;220000;110000_Station_Dauersberg/RConn4 -- L_152403632/LConn1
  T_152403632_380000;220000;110000_Station_Dauersberg/RConn5 -- L_152403632/LConn2
  T_152403632_380000;220000;110000_Station_Dauersberg/RConn6 -- L_152403632/LConn3
  T_92165128_380000;110000_Station_Linde/RConn1 -- L_92165128/LConn1
  T_92165128_380000;110000_Station_Linde/RConn2 -- L_92165128/LConn2
  T_92165128_380000;110000_Station_Linde/RConn3 -- L_92165128/LConn3
  T_32731290_220000;110000_Karlsruhe_West/RConn1 -- L_32731290/LConn1
  T_32731290_220000;110000_Karlsruhe_West/RConn2 -- L_32731290/LConn2
  T_32731290_220000;110000_Karlsruhe_West/RConn3 -- L_32731290/LConn3
  T_234950814__/RConn1 -- L_234950814/LConn1
  T_234950814__/RConn2 -- L_234950814/LConn2
  T_234950814__/RConn3 -- L_234950814/LConn3
  T_26927264_380000;110000_Station_Paffendorf/RConn1 -- L_26927264/LConn1
  T_26927264_380000;110000_Station_Paffendorf/RConn2 -- L_26927264/LConn2
  T_26927264_380000;110000_Station_Paffendorf/RConn3 -- L_26927264/LConn3
  T_23406775_380000;110000_Pulgar/RConn1 -- L_23406775/LConn1
  T_23406775_380000;110000_Pulgar/RConn2 -- L_23406775/LConn2
  T_23406775_380000;110000_Pulgar/RConn3 -- L_23406775/LConn3
  T_143882655_380000;220000;110000_Umspannwerk_Vieselbach/RConn4 -- L_143882655/LConn1
  T_143882655_380000;220000;110000_Umspannwerk_Vieselbach/RConn5 -- L_143882655/LConn2
  T_143882655_380000;220000;110000_Umspannwerk_Vieselbach/RConn6 -- L_143882655/LConn3
  T_32843531_380000;220000;110000_Eula/RConn4 -- L_32843531/LConn1
  T_32843531_380000;220000;110000_Eula/RConn5 -- L_32843531/LConn2
  T_32843531_380000;220000;110000_Eula/RConn6 -- L_32843531/LConn3
  T_31131325_380000;110000_380kV_Umspannwerk_Grünkraut/RConn1 -- L_31131325/LConn1
  T_31131325_380000;110000_380kV_Umspannwerk_Grünkraut/RConn2 -- L_31131325/LConn2
  T_31131325_380000;110000_380kV_Umspannwerk_Grünkraut/RConn3 -- L_31131325/LConn3
  T_154110133_380000_/RConn1 -- L_154110133/LConn1
  T_154110133_380000_/RConn2 -- L_154110133/LConn2
  T_154110133_380000_/RConn3 -- L_154110133/LConn3
  T_154110135_380000_Philippsburg_380_kV/RConn1 -- L_154110135/LConn1
  T_154110135_380000_Philippsburg_380_kV/RConn2 -- L_154110135/LConn2
  T_154110135_380000_Philippsburg_380_kV/RConn3 -- L_154110135/LConn3
  T_90109302_220000_UA_Obergraben/RConn1 -- L_90109302/LConn1
  T_90109302_220000_UA_Obergraben/RConn2 -- L_90109302/LConn2
  T_90109302_220000_UA_Obergraben/RConn3 -- L_90109302/LConn3
  T_28397771_220000;110000_UW_Veltheim/RConn1 -- L_28397771/LConn1
  T_28397771_220000;110000_UW_Veltheim/RConn2 -- L_28397771/LConn2
  T_28397771_220000;110000_UW_Veltheim/RConn3 -- L_28397771/LConn3
  T_23135618_220000;110000_Umspannwerk_Meißen/RConn1 -- L_23135618/LConn1
  T_23135618_220000;110000_Umspannwerk_Meißen/RConn2 -- L_23135618/LConn2
  T_23135618_220000;110000_Umspannwerk_Meißen/RConn3 -- L_23135618/LConn3
  T_26611458_220000;110000_Umspannwerk_Bielefeld_Ost/RConn1 -- L_26611458/LConn1
  T_26611458_220000;110000_Umspannwerk_Bielefeld_Ost/RConn2 -- L_26611458/LConn2
  T_26611458_220000;110000_Umspannwerk_Bielefeld_Ost/RConn3 -- L_26611458/LConn3
  T_24264701_380000;220000;110000_Umspannwerk_Bechterdissen/RConn4 -- L_24264701/LConn1
  T_24264701_380000;220000;110000_Umspannwerk_Bechterdissen/RConn5 -- L_24264701/LConn2
  T_24264701_380000;220000;110000_Umspannwerk_Bechterdissen/RConn6 -- L_24264701/LConn3
  T_288305056_220000;110000_Umspannwerk_Lage/RConn1 -- L_288305056/LConn1
  T_288305056_220000;110000_Umspannwerk_Lage/RConn2 -- L_288305056/LConn2
  T_288305056_220000;110000_Umspannwerk_Lage/RConn3 -- L_288305056/LConn3
  T_149256409_380000;110000_Umspannwerk_Altenfeld/RConn1 -- L_149256409/LConn1
  T_149256409_380000;110000_Umspannwerk_Altenfeld/RConn2 -- L_149256409/LConn2
  T_149256409_380000;110000_Umspannwerk_Altenfeld/RConn3 -- L_149256409/LConn3
  T_25746125_380000_Pumpspeicherwerk_Goldisthal/RConn1 -- L_25746125/LConn1
  T_25746125_380000_Pumpspeicherwerk_Goldisthal/RConn2 -- L_25746125/LConn2
  T_25746125_380000_Pumpspeicherwerk_Goldisthal/RConn3 -- L_25746125/LConn3
  T_128277645_380000;220000;110000_Umspannwerk_Remptendorf/RConn4 -- L_128277645/LConn1
  T_128277645_380000;220000;110000_Umspannwerk_Remptendorf/RConn5 -- L_128277645/LConn2
  T_128277645_380000;220000;110000_Umspannwerk_Remptendorf/RConn6 -- L_128277645/LConn3
  T_150200540_220000_Kraftwerkschaltanlage_Ibbenbüren/RConn1 -- L_150200540/LConn1
  T_150200540_220000_Kraftwerkschaltanlage_Ibbenbüren/RConn2 -- L_150200540/LConn2
  T_150200540_220000_Kraftwerkschaltanlage_Ibbenbüren/RConn3 -- L_150200540/LConn3
  T_37554416_220000;110000_Station_Hamborn/RConn1 -- L_37554416/LConn1
  T_37554416_220000;110000_Station_Hamborn/RConn2 -- L_37554416/LConn2
  T_37554416_220000;110000_Station_Hamborn/RConn3 -- L_37554416/LConn3
  T_35833592_220000_/RConn1 -- L_35833592/LConn1
  T_35833592_220000_/RConn2 -- L_35833592/LConn2
  T_35833592_220000_/RConn3 -- L_35833592/LConn3
  T_35818137_380000;220000;110000_Station_Beeck/RConn1 -- L_35818137/LConn1
  T_35818137_380000;220000;110000_Station_Beeck/RConn2 -- L_35818137/LConn2
  T_35818137_380000;220000;110000_Station_Beeck/RConn3 -- L_35818137/LConn3
  T_24462426_380000;220000;110000_Station_Niederrhein/RConn4 -- L_24462426/LConn1
  T_24462426_380000;220000;110000_Station_Niederrhein/RConn5 -- L_24462426/LConn2
  T_24462426_380000;220000;110000_Station_Niederrhein/RConn6 -- L_24462426/LConn3
  T_46852069_220000;110000_Station_Handbach/RConn1 -- L_46852069/LConn1
  T_46852069_220000;110000_Station_Handbach/RConn2 -- L_46852069/LConn2
  T_46852069_220000;110000_Station_Handbach/RConn3 -- L_46852069/LConn3
  T_25032036_220000;110000_Styrum/RConn1 -- L_25032036/LConn1
  T_25032036_220000;110000_Styrum/RConn2 -- L_25032036/LConn2
  T_25032036_220000;110000_Styrum/RConn3 -- L_25032036/LConn3
  T_137197826_380000;220000;110000_Neuenhagen/RConn4 -- L_137197826/LConn1
  T_137197826_380000;220000;110000_Neuenhagen/RConn5 -- L_137197826/LConn2
  T_137197826_380000;220000;110000_Neuenhagen/RConn6 -- L_137197826/LConn3
  T_52983550_380000;110000_Eisenhüttenstadt/RConn1 -- L_52983550/LConn1
  T_52983550_380000;110000_Eisenhüttenstadt/RConn2 -- L_52983550/LConn2
  T_52983550_380000;110000_Eisenhüttenstadt/RConn3 -- L_52983550/LConn3
  T_23025610_380000;110000_Umspannwerk_Preilack/RConn1 -- L_23025610/LConn1
  T_23025610_380000;110000_Umspannwerk_Preilack/RConn2 -- L_23025610/LConn2
  T_23025610_380000;110000_Umspannwerk_Preilack/RConn3 -- L_23025610/LConn3
  T_20562114_380000;110000_Umspannwerk_Malchow/RConn1 -- L_20562114/LConn1
  T_20562114_380000;110000_Umspannwerk_Malchow/RConn2 -- L_20562114/LConn2
  T_20562114_380000;110000_Umspannwerk_Malchow/RConn3 -- L_20562114/LConn3
  T_22973070_380000;220000;110000_Umspannwerk_Marzahn/RConn4 -- L_22973070/LConn1
  T_22973070_380000;220000;110000_Umspannwerk_Marzahn/RConn5 -- L_22973070/LConn2
  T_22973070_380000;220000;110000_Umspannwerk_Marzahn/RConn6 -- L_22973070/LConn3
  T_29331499_380000;220000;110000_Thyrow/RConn4 -- L_29331499/LConn1
  T_29331499_380000;220000;110000_Thyrow/RConn5 -- L_29331499/LConn2
  T_29331499_380000;220000;110000_Thyrow/RConn6 -- L_29331499/LConn3
  T_27149550_380000;220000;110000_Wustermark/RConn4 -- L_27149550/LConn1
  T_27149550_380000;220000;110000_Wustermark/RConn5 -- L_27149550/LConn2
  T_27149550_380000;220000;110000_Wustermark/RConn6 -- L_27149550/LConn3
  T_22973052_220000;110000_Umspannwerk_Wuhlheide/RConn1 -- L_22973052/LConn1
  T_22973052_220000;110000_Umspannwerk_Wuhlheide/RConn2 -- L_22973052/LConn2
  T_22973052_220000;110000_Umspannwerk_Wuhlheide/RConn3 -- L_22973052/LConn3
  T_26474759_380000;110000_Umspannwerk_Helmstedt/RConn1 -- L_26474759/LConn1
  T_26474759_380000;110000_Umspannwerk_Helmstedt/RConn2 -- L_26474759/LConn2
  T_26474759_380000;110000_Umspannwerk_Helmstedt/RConn3 -- L_26474759/LConn3
  T_199382606__/RConn1 -- L_199382606/LConn1
  T_199382606__/RConn2 -- L_199382606/LConn2
  T_199382606__/RConn3 -- L_199382606/LConn3
  T_151765495_220000_Götzdorf/RConn1 -- L_151765495/LConn1
  T_151765495_220000_Götzdorf/RConn2 -- L_151765495/LConn2
  T_151765495_220000_Götzdorf/RConn3 -- L_151765495/LConn3
  T_25306938_220000;110000_Kummerfeld/RConn1 -- L_25306938/LConn1
  T_25306938_220000;110000_Kummerfeld/RConn2 -- L_25306938/LConn2
  T_25306938_220000;110000_Kummerfeld/RConn3 -- L_25306938/LConn3
  T_25557259__/RConn1 -- L_25557259/LConn1
  T_25557259__/RConn2 -- L_25557259/LConn2
  T_25557259__/RConn3 -- L_25557259/LConn3
  T_143854536_380000;110000_Umspannwerk_Kupferzell/RConn1 -- L_143854536/LConn1
  T_143854536_380000;110000_Umspannwerk_Kupferzell/RConn2 -- L_143854536/LConn2
  T_143854536_380000;110000_Umspannwerk_Kupferzell/RConn3 -- L_143854536/LConn3
  T_145002769_380000;110000_Umspannwerk_Höpfingen/RConn1 -- L_145002769/LConn1
  T_145002769_380000;110000_Umspannwerk_Höpfingen/RConn2 -- L_145002769/LConn2
  T_145002769_380000;110000_Umspannwerk_Höpfingen/RConn3 -- L_145002769/LConn3
  T_153328698_380000_Gemeinschaftskraftwerk_Neckarwestheim_2/RConn1 -- L_153328698/LConn1
  T_153328698_380000_Gemeinschaftskraftwerk_Neckarwestheim_2/RConn2 -- L_153328698/LConn2
  T_153328698_380000_Gemeinschaftskraftwerk_Neckarwestheim_2/RConn3 -- L_153328698/LConn3
  T_169244940_380000_Station_Kelsterbach/RConn1 -- L_169244940/LConn1
  T_169244940_380000_Station_Kelsterbach/RConn2 -- L_169244940/LConn2
  T_169244940_380000_Station_Kelsterbach/RConn3 -- L_169244940/LConn3
  T_55730023_380000_Kabeleinführung_380_kV/RConn1 -- L_55730023/LConn1
  T_55730023_380000_Kabeleinführung_380_kV/RConn2 -- L_55730023/LConn2
  T_55730023_380000_Kabeleinführung_380_kV/RConn3 -- L_55730023/LConn3
  T_29417741_220000_Umspannwerk_Regensburg/RConn1 -- L_29417741/LConn1
  T_29417741_220000_Umspannwerk_Regensburg/RConn2 -- L_29417741/LConn2
  T_29417741_220000_Umspannwerk_Regensburg/RConn3 -- L_29417741/LConn3
  T_28729619_380000_Umspannwerk_Schönewalde/RConn1 -- L_28729619/LConn1
  T_28729619_380000_Umspannwerk_Schönewalde/RConn2 -- L_28729619/LConn2
  T_28729619_380000_Umspannwerk_Schönewalde/RConn3 -- L_28729619/LConn3
  T_25526912_380000;110000_Umspannwerk_Marke/RConn1 -- L_25526912/LConn1
  T_25526912_380000;110000_Umspannwerk_Marke/RConn2 -- L_25526912/LConn2
  T_25526912_380000;110000_Umspannwerk_Marke/RConn3 -- L_25526912/LConn3
  T_29713902_380000;110000_Umspannwerk_Lauchstädt/RConn1 -- L_29713902/LConn1
  T_29713902_380000;110000_Umspannwerk_Lauchstädt/RConn2 -- L_29713902/LConn2
  T_29713902_380000;110000_Umspannwerk_Lauchstädt/RConn3 -- L_29713902/LConn3
  T_156683994_380000;110000_Umspannwerk_Ragow/RConn1 -- L_156683994/LConn1
  T_156683994_380000;110000_Umspannwerk_Ragow/RConn2 -- L_156683994/LConn2
  T_156683994_380000;110000_Umspannwerk_Ragow/RConn3 -- L_156683994/LConn3
  T_53378027_380000;110000_Umspannwerk_Lechhausen;_Übernahmestation_Lechhausen/RConn1 -- L_53378027/LConn1
  T_53378027_380000;110000_Umspannwerk_Lechhausen;_Übernahmestation_Lechhausen/RConn2 -- L_53378027/LConn2
  T_53378027_380000;110000_Umspannwerk_Lechhausen;_Übernahmestation_Lechhausen/RConn3 -- L_53378027/LConn3
  T_24652261_380000_Station_Meitingen/RConn1 -- L_24652261/LConn1
  T_24652261_380000_Station_Meitingen/RConn2 -- L_24652261/LConn2
  T_24652261_380000_Station_Meitingen/RConn3 -- L_24652261/LConn3
  T_42097854_380000;110000_Station_Osburg/RConn1 -- L_42097854/LConn1
  T_42097854_380000;110000_Station_Osburg/RConn2 -- L_42097854/LConn2
  T_42097854_380000;110000_Station_Osburg/RConn3 -- L_42097854/LConn3
  T_156973363_220000_Station_Welper/RConn1 -- L_156973363/LConn1
  T_156973363_220000_Station_Welper/RConn2 -- L_156973363/LConn2
  T_156973363_220000_Station_Welper/RConn3 -- L_156973363/LConn3
  T_86163350_220000_UW_Stahlwerk_ThyssenKrupp_Nirosta/RConn1 -- L_86163350/LConn1
  T_86163350_220000_UW_Stahlwerk_ThyssenKrupp_Nirosta/RConn2 -- L_86163350/LConn2
  T_86163350_220000_UW_Stahlwerk_ThyssenKrupp_Nirosta/RConn3 -- L_86163350/LConn3
  T_153334076__/RConn1 -- L_153334076/LConn1
  T_153334076__/RConn2 -- L_153334076/LConn2
  T_153334076__/RConn3 -- L_153334076/LConn3
  T_35102433_220000;110000_Magdeburg_(50Hertz)/RConn1 -- L_35102433/LConn1
  T_35102433_220000;110000_Magdeburg_(50Hertz)/RConn2 -- L_35102433/LConn2
  T_35102433_220000;110000_Magdeburg_(50Hertz)/RConn3 -- L_35102433/LConn3
  T_35137205_220000;110000_Umspannwerk_Förderstedt/RConn1 -- L_35137205/LConn1
  T_35137205_220000;110000_Umspannwerk_Förderstedt/RConn2 -- L_35137205/LConn2
  T_35137205_220000;110000_Umspannwerk_Förderstedt/RConn3 -- L_35137205/LConn3
  T_91086220_220000_Umspannwerk_Simbach/RConn1 -- L_91086220/LConn1
  T_91086220_220000_Umspannwerk_Simbach/RConn2 -- L_91086220/LConn2
  T_91086220_220000_Umspannwerk_Simbach/RConn3 -- L_91086220/LConn3
  T_24976300_380000;220000;110000_Umspannwerk_Pleinting/RConn4 -- L_24976300/LConn1
  T_24976300_380000;220000;110000_Umspannwerk_Pleinting/RConn5 -- L_24976300/LConn2
  T_24976300_380000;220000;110000_Umspannwerk_Pleinting/RConn6 -- L_24976300/LConn3
  T_77694901_220000;110000_Umspannwerk_Altheim/RConn1 -- L_77694901/LConn1
  T_77694901_220000;110000_Umspannwerk_Altheim/RConn2 -- L_77694901/LConn2
  T_77694901_220000;110000_Umspannwerk_Altheim/RConn3 -- L_77694901/LConn3
  T_93278553_220000;110000_Station_Edelstahl_Krefeld/RConn1 -- L_93278553/LConn1
  T_93278553_220000;110000_Station_Edelstahl_Krefeld/RConn2 -- L_93278553/LConn2
  T_93278553_220000;110000_Station_Edelstahl_Krefeld/RConn3 -- L_93278553/LConn3
  T_24815262_380000;220000;110000_Station_Dülken/RConn1 -- L_24815262/LConn1
  T_24815262_380000;220000;110000_Station_Dülken/RConn2 -- L_24815262/LConn2
  T_24815262_380000;220000;110000_Station_Dülken/RConn3 -- L_24815262/LConn3
  T_23380800_380000;220000;110000_Station_Utfort/RConn4 -- L_23380800/LConn1
  T_23380800_380000;220000;110000_Station_Utfort/RConn5 -- L_23380800/LConn2
  T_23380800_380000;220000;110000_Station_Utfort/RConn6 -- L_23380800/LConn3
  T_24479984_220000;110000_Uerdingen/RConn1 -- L_24479984/LConn1
  T_24479984_220000;110000_Uerdingen/RConn2 -- L_24479984/LConn2
  T_24479984_220000;110000_Uerdingen/RConn3 -- L_24479984/LConn3
  T_74893659_380000;110000_HGÜ_Baltic_Cable___Stromrichterstation_Herrenwyk/RConn1 -- L_74893659/LConn1
  T_74893659_380000;110000_HGÜ_Baltic_Cable___Stromrichterstation_Herrenwyk/RConn2 -- L_74893659/LConn2
  T_74893659_380000;110000_HGÜ_Baltic_Cable___Stromrichterstation_Herrenwyk/RConn3 -- L_74893659/LConn3
  T_74893662_380000;220000;110000_Umspannwerk_Siems/RConn1 -- L_74893662/LConn1
  T_74893662_380000;220000;110000_Umspannwerk_Siems/RConn2 -- L_74893662/LConn2
  T_74893662_380000;220000;110000_Umspannwerk_Siems/RConn3 -- L_74893662/LConn3
  T_156398578__Station_Ronsdorf/RConn1 -- L_156398578/LConn1
  T_156398578__Station_Ronsdorf/RConn2 -- L_156398578/LConn2
  T_156398578__Station_Ronsdorf/RConn3 -- L_156398578/LConn3
  T_22761692_220000;110000_UW_Fühlingen/RConn1 -- L_22761692/LConn1
  T_22761692_220000;110000_UW_Fühlingen/RConn2 -- L_22761692/LConn2
  T_22761692_220000;110000_UW_Fühlingen/RConn3 -- L_22761692/LConn3
  T_22764922_220000;110000_Station_Dhünnaue/RConn1 -- L_22764922/LConn1
  T_22764922_220000;110000_Station_Dhünnaue/RConn2 -- L_22764922/LConn2
  T_22764922_220000;110000_Station_Dhünnaue/RConn3 -- L_22764922/LConn3
  T_49577448_380000;220000_Station_Sankt_Peter_380_kV/RConn1 -- L_49577448/LConn1
  T_49577448_380000;220000_Station_Sankt_Peter_380_kV/RConn2 -- L_49577448/LConn2
  T_49577448_380000;220000_Station_Sankt_Peter_380_kV/RConn3 -- L_49577448/LConn3
  T_106096507_380000;110000_Station_Ohligs/RConn1 -- L_106096507/LConn1
  T_106096507_380000;110000_Station_Ohligs/RConn2 -- L_106096507/LConn2
  T_106096507_380000;110000_Station_Ohligs/RConn3 -- L_106096507/LConn3
  T_42799487_380000;110000_Station_Arpe/RConn1 -- L_42799487/LConn1
  T_42799487_380000;110000_Station_Arpe/RConn2 -- L_42799487/LConn2
  T_42799487_380000;110000_Station_Arpe/RConn3 -- L_42799487/LConn3
  T_42797575_380000;110000_Station_Nehden/RConn1 -- L_42797575/LConn1
  T_42797575_380000;110000_Station_Nehden/RConn2 -- L_42797575/LConn2
  T_42797575_380000;110000_Station_Nehden/RConn3 -- L_42797575/LConn3
  T_77179271_380000_Station_Osterath/RConn1 -- L_77179271/LConn1
  T_77179271_380000_Station_Osterath/RConn2 -- L_77179271/LConn2
  T_77179271_380000_Station_Osterath/RConn3 -- L_77179271/LConn3
  T_207488608__/RConn1 -- L_207488608/LConn1
  T_207488608__/RConn2 -- L_207488608/LConn2
  T_207488608__/RConn3 -- L_207488608/LConn3
  T_25044557_380000_Station_Rath/RConn1 -- L_25044557/LConn1
  T_25044557_380000_Station_Rath/RConn2 -- L_25044557/LConn2
  T_25044557_380000_Station_Rath/RConn3 -- L_25044557/LConn3
  T_157806991_380000_Umspannwerk_Bärwalde/RConn1 -- L_157806991/LConn1
  T_157806991_380000_Umspannwerk_Bärwalde/RConn2 -- L_157806991/LConn2
  T_157806991_380000_Umspannwerk_Bärwalde/RConn3 -- L_157806991/LConn3
  T_157328339_380000;110000_Umspannwerk_Streumen/RConn1 -- L_157328339/LConn1
  T_157328339_380000;110000_Umspannwerk_Streumen/RConn2 -- L_157328339/LConn2
  T_157328339_380000;110000_Umspannwerk_Streumen/RConn3 -- L_157328339/LConn3
  T_30164703_380000;110000_Graustein/RConn1 -- L_30164703/LConn1
  T_30164703_380000;110000_Graustein/RConn2 -- L_30164703/LConn2
  T_30164703_380000;110000_Graustein/RConn3 -- L_30164703/LConn3
  T_157807291_380000;110000_Umspannwerk_Schmölln/RConn1 -- L_157807291/LConn1
  T_157807291_380000;110000_Umspannwerk_Schmölln/RConn2 -- L_157807291/LConn2
  T_157807291_380000;110000_Umspannwerk_Schmölln/RConn3 -- L_157807291/LConn3
  T_35176751_380000;110000_Audorf/RConn1 -- L_35176751/LConn1
  T_35176751_380000;110000_Audorf/RConn2 -- L_35176751/LConn2
  T_35176751_380000;110000_Audorf/RConn3 -- L_35176751/LConn3
  T_301158539_380000;110000;20000_Umspannwerk_Jardelund/RConn1 -- L_301158539/LConn1
  T_301158539_380000;110000;20000_Umspannwerk_Jardelund/RConn2 -- L_301158539/LConn2
  T_301158539_380000;110000;20000_Umspannwerk_Jardelund/RConn3 -- L_301158539/LConn3
  T_87952821_380000;220000;110000;20000_Flensburg/RConn4 -- L_87952821/LConn1
  T_87952821_380000;220000;110000;20000_Flensburg/RConn5 -- L_87952821/LConn2
  T_87952821_380000;220000;110000;20000_Flensburg/RConn6 -- L_87952821/LConn3
  T_159326655_220000;110000_Obrigheim/RConn1 -- L_159326655/LConn1
  T_159326655_220000;110000_Obrigheim/RConn2 -- L_159326655/LConn2
  T_159326655_220000;110000_Obrigheim/RConn3 -- L_159326655/LConn3
  T_104878489_220000;110000_Umspannwerk_Kraftwerk_Emden/RConn1 -- L_104878489/LConn1
  T_104878489_220000;110000_Umspannwerk_Kraftwerk_Emden/RConn2 -- L_104878489/LConn2
  T_104878489_220000;110000_Umspannwerk_Kraftwerk_Emden/RConn3 -- L_104878489/LConn3
  T_34835258_220000;110000_Emden_Borßum/RConn1 -- L_34835258/LConn1
  T_34835258_220000;110000_Emden_Borßum/RConn2 -- L_34835258/LConn2
  T_34835258_220000;110000_Emden_Borßum/RConn3 -- L_34835258/LConn3
  T_157164284_220000_Wolkramshausen_(220_kV)/RConn1 -- L_157164284/LConn1
  T_157164284_220000_Wolkramshausen_(220_kV)/RConn2 -- L_157164284/LConn2
  T_157164284_220000_Wolkramshausen_(220_kV)/RConn3 -- L_157164284/LConn3
  T_29309786_380000;110000_Mecklar/RConn1 -- L_29309786/LConn1
  T_29309786_380000;110000_Mecklar/RConn2 -- L_29309786/LConn2
  T_29309786_380000;110000_Mecklar/RConn3 -- L_29309786/LConn3
  T_154418450_380000;110000_Eisenach/RConn1 -- L_154418450/LConn1
  T_154418450_380000;110000_Eisenach/RConn2 -- L_154418450/LConn2
  T_154418450_380000;110000_Eisenach/RConn3 -- L_154418450/LConn3
  T_148211527_380000;110000_Großschwabhausen/RConn1 -- L_148211527/LConn1
  T_148211527_380000;110000_Großschwabhausen/RConn2 -- L_148211527/LConn2
  T_148211527_380000;110000_Großschwabhausen/RConn3 -- L_148211527/LConn3
  T_145486242__/RConn1 -- L_145486242/LConn1
  T_145486242__/RConn2 -- L_145486242/LConn2
  T_145486242__/RConn3 -- L_145486242/LConn3
  T_24267175_220000;110000_Umspannanlage_Frimmersdorf_I/RConn1 -- L_24267175/LConn1
  T_24267175_220000;110000_Umspannanlage_Frimmersdorf_I/RConn2 -- L_24267175/LConn2
  T_24267175_220000;110000_Umspannanlage_Frimmersdorf_I/RConn3 -- L_24267175/LConn3
  T_151507370_220000_/RConn1 -- L_151507370/LConn1
  T_151507370_220000_/RConn2 -- L_151507370/LConn2
  T_151507370_220000_/RConn3 -- L_151507370/LConn3
  T_50643382_220000_Cloppenburg_220_kV/RConn1 -- L_50643382/LConn1
  T_50643382_220000_Cloppenburg_220_kV/RConn2 -- L_50643382/LConn2
  T_50643382_220000_Cloppenburg_220_kV/RConn3 -- L_50643382/LConn3
  T_173178563_220000;110000_Conneforde_110_220_kV/RConn1 -- L_173178563/LConn1
  T_173178563_220000;110000_Conneforde_110_220_kV/RConn2 -- L_173178563/LConn2
  T_173178563_220000;110000_Conneforde_110_220_kV/RConn3 -- L_173178563/LConn3
  T_68532663_220000;110000_Umspannwerk_Krün/RConn1 -- L_68532663/LConn1
  T_68532663_220000;110000_Umspannwerk_Krün/RConn2 -- L_68532663/LConn2
  T_68532663_220000;110000_Umspannwerk_Krün/RConn3 -- L_68532663/LConn3
  T_24237879_220000;110000_Umspannwerk_Oberbrunn/RConn1 -- L_24237879/LConn1
  T_24237879_220000;110000_Umspannwerk_Oberbrunn/RConn2 -- L_24237879/LConn2
  T_24237879_220000;110000_Umspannwerk_Oberbrunn/RConn3 -- L_24237879/LConn3
  T_39229429_220000;110000_Station_Hesseln/RConn1 -- L_39229429/LConn1
  T_39229429_220000;110000_Station_Hesseln/RConn2 -- L_39229429/LConn2
  T_39229429_220000;110000_Station_Hesseln/RConn3 -- L_39229429/LConn3
  T_32993727_220000;110000_KW_Niederaußem/RConn1 -- L_32993727/LConn1
  T_32993727_220000;110000_KW_Niederaußem/RConn2 -- L_32993727/LConn2
  T_32993727_220000;110000_KW_Niederaußem/RConn3 -- L_32993727/LConn3
  T_133342285_220000;110000_Zolling___Irsching/RConn1 -- L_133342285/LConn1
  T_133342285_220000;110000_Zolling___Irsching/RConn2 -- L_133342285/LConn2
  T_133342285_220000;110000_Zolling___Irsching/RConn3 -- L_133342285/LConn3
  T_75865676_220000_Umspannwerk_Marienberg/RConn1 -- L_75865676/LConn1
  T_75865676_220000_Umspannwerk_Marienberg/RConn2 -- L_75865676/LConn2
  T_75865676_220000_Umspannwerk_Marienberg/RConn3 -- L_75865676/LConn3
  T_35833442_220000_/RConn1 -- L_35833442/LConn1
  T_35833442_220000_/RConn2 -- L_35833442/LConn2
  T_35833442_220000_/RConn3 -- L_35833442/LConn3
  T_158253525_220000;110000_Umspannwerk_Paderborn_Süd/RConn1 -- L_158253525/LConn1
  T_158253525_220000;110000_Umspannwerk_Paderborn_Süd/RConn2 -- L_158253525/LConn2
  T_158253525_220000;110000_Umspannwerk_Paderborn_Süd/RConn3 -- L_158253525/LConn3
  T_30132758_380000;110000_Teufelsbruch/RConn1 -- L_30132758/LConn1
  T_30132758_380000;110000_Teufelsbruch/RConn2 -- L_30132758/LConn2
  T_30132758_380000;110000_Teufelsbruch/RConn3 -- L_30132758/LConn3
  T_32690742_380000;110000_Umspannwerk_Klostermansfeld/RConn1 -- L_32690742/LConn1
  T_32690742_380000;110000_Umspannwerk_Klostermansfeld/RConn2 -- L_32690742/LConn2
  T_32690742_380000;110000_Umspannwerk_Klostermansfeld/RConn3 -- L_32690742/LConn3
  T_24414688_220000;110000_Station_Wambel/RConn1 -- L_24414688/LConn1
  T_24414688_220000;110000_Station_Wambel/RConn2 -- L_24414688/LConn2
  T_24414688_220000;110000_Station_Wambel/RConn3 -- L_24414688/LConn3
  T_24858617_220000_Ratsbusch/RConn1 -- L_24858617/LConn1
  T_24858617_220000_Ratsbusch/RConn2 -- L_24858617/LConn2
  T_24858617_220000_Ratsbusch/RConn3 -- L_24858617/LConn3
  T_88945213_380000_Umspannwerk_Gundelfingen/RConn1 -- L_88945213/LConn1
  T_88945213_380000_Umspannwerk_Gundelfingen/RConn2 -- L_88945213/LConn2
  T_88945213_380000_Umspannwerk_Gundelfingen/RConn3 -- L_88945213/LConn3
  T_76246159_380000;110000_Umspannwerk_Meitingen/RConn1 -- L_76246159/LConn1
  T_76246159_380000;110000_Umspannwerk_Meitingen/RConn2 -- L_76246159/LConn2
  T_76246159_380000;110000_Umspannwerk_Meitingen/RConn3 -- L_76246159/LConn3
  T_22879599_220000;110000_Umspannwerk_Großdalzig/RConn1 -- L_22879599/LConn1
  T_22879599_220000;110000_Umspannwerk_Großdalzig/RConn2 -- L_22879599/LConn2
  T_22879599_220000;110000_Umspannwerk_Großdalzig/RConn3 -- L_22879599/LConn3
  T_229500139_220000_DOW/RConn1 -- L_229500139/LConn1
  T_229500139_220000_DOW/RConn2 -- L_229500139/LConn2
  T_229500139_220000_DOW/RConn3 -- L_229500139/LConn3
  T_30040568_380000;110000_Görries/RConn1 -- L_30040568/LConn1
  T_30040568_380000;110000_Görries/RConn2 -- L_30040568/LConn2
  T_30040568_380000;110000_Görries/RConn3 -- L_30040568/LConn3
  T_23366603_380000;110000_Krümmel/RConn1 -- L_23366603/LConn1
  T_23366603_380000;110000_Krümmel/RConn2 -- L_23366603/LConn2
  T_23366603_380000;110000_Krümmel/RConn3 -- L_23366603/LConn3
  T_234171369_380000_Wessin/RConn1 -- L_234171369/LConn1
  T_234171369_380000_Wessin/RConn2 -- L_234171369/LConn2
  T_234171369_380000_Wessin/RConn3 -- L_234171369/LConn3
  T_41232144_380000;110000_Umspannwerk_Twistetal/RConn1 -- L_41232144/LConn1
  T_41232144_380000;110000_Umspannwerk_Twistetal/RConn2 -- L_41232144/LConn2
  T_41232144_380000;110000_Umspannwerk_Twistetal/RConn3 -- L_41232144/LConn3
  T_25943440_380000;110000_Umspannwerk_Elsen/RConn1 -- L_25943440/LConn1
  T_25943440_380000;110000_Umspannwerk_Elsen/RConn2 -- L_25943440/LConn2
  T_25943440_380000;110000_Umspannwerk_Elsen/RConn3 -- L_25943440/LConn3
  T_163093653_220000;110000_Mannheim/RConn1 -- L_163093653/LConn1
  T_163093653_220000;110000_Mannheim/RConn2 -- L_163093653/LConn2
  T_163093653_220000;110000_Mannheim/RConn3 -- L_163093653/LConn3
  T_160929097_220000;110000_Umspannwerk_Weinheim/RConn1 -- L_160929097/LConn1
  T_160929097_220000;110000_Umspannwerk_Weinheim/RConn2 -- L_160929097/LConn2
  T_160929097_220000;110000_Umspannwerk_Weinheim/RConn3 -- L_160929097/LConn3
  T_154729020_220000;110000_Umspannwerk_Altlußheim/RConn1 -- L_154729020/LConn1
  T_154729020_220000;110000_Umspannwerk_Altlußheim/RConn2 -- L_154729020/LConn2
  T_154729020_220000;110000_Umspannwerk_Altlußheim/RConn3 -- L_154729020/LConn3
  T_152018146_380000_Mittelbexbach/RConn1 -- L_152018146/LConn1
  T_152018146_380000_Mittelbexbach/RConn2 -- L_152018146/LConn2
  T_152018146_380000_Mittelbexbach/RConn3 -- L_152018146/LConn3
  T_32966636_220000;110000_220_kV_Umspannwerk_Birkenfeld/RConn1 -- L_32966636/LConn1
  T_32966636_220000;110000_220_kV_Umspannwerk_Birkenfeld/RConn2 -- L_32966636/LConn2
  T_32966636_220000;110000_220_kV_Umspannwerk_Birkenfeld/RConn3 -- L_32966636/LConn3
  T_32725957_220000;110000_Umspannwerk_Oberwald/RConn1 -- L_32725957/LConn1
  T_32725957_220000;110000_Umspannwerk_Oberwald/RConn2 -- L_32725957/LConn2
  T_32725957_220000;110000_Umspannwerk_Oberwald/RConn3 -- L_32725957/LConn3
  T_87653464_220000;110000_220_kV_Umspannwerk_Eichstetten/RConn1 -- L_87653464/LConn1
  T_87653464_220000;110000_220_kV_Umspannwerk_Eichstetten/RConn2 -- L_87653464/LConn2
  T_87653464_220000;110000_220_kV_Umspannwerk_Eichstetten/RConn3 -- L_87653464/LConn3
  T_24280460_380000;110000_Station_Nordlicht/RConn1 -- L_24280460/LConn1
  T_24280460_380000;110000_Station_Nordlicht/RConn2 -- L_24280460/LConn2
  T_24280460_380000;110000_Station_Nordlicht/RConn3 -- L_24280460/LConn3
  T_26291794_380000;110000_Station_Rosenblumendelle/RConn1 -- L_26291794/LConn1
  T_26291794_380000;110000_Station_Rosenblumendelle/RConn2 -- L_26291794/LConn2
  T_26291794_380000;110000_Station_Rosenblumendelle/RConn3 -- L_26291794/LConn3
  T_78441561_380000;110000_Umspannwerk_Plattling/RConn1 -- L_78441561/LConn1
  T_78441561_380000;110000_Umspannwerk_Plattling/RConn2 -- L_78441561/LConn2
  T_78441561_380000;110000_Umspannwerk_Plattling/RConn3 -- L_78441561/LConn3
  T_24462228_220000;110000_Station_Ossenberg/RConn1 -- L_24462228/LConn1
  T_24462228_220000;110000_Station_Ossenberg/RConn2 -- L_24462228/LConn2
  T_24462228_220000;110000_Station_Ossenberg/RConn3 -- L_24462228/LConn3
  T_23084417_220000;110000_Station_Pfalzdorf/RConn1 -- L_23084417/LConn1
  T_23084417_220000;110000_Station_Pfalzdorf/RConn2 -- L_23084417/LConn2
  T_23084417_220000;110000_Station_Pfalzdorf/RConn3 -- L_23084417/LConn3
  T_33042984_220000;110000_TenneT_TSO_GmbH___Betriebszentrum_Lehrte/RConn1 -- L_33042984/LConn1
  T_33042984_220000;110000_TenneT_TSO_GmbH___Betriebszentrum_Lehrte/RConn2 -- L_33042984/LConn2
  T_33042984_220000;110000_TenneT_TSO_GmbH___Betriebszentrum_Lehrte/RConn3 -- L_33042984/LConn3
  T_160093341_220000_Erzhausen/RConn1 -- L_160093341/LConn1
  T_160093341_220000_Erzhausen/RConn2 -- L_160093341/LConn2
  T_160093341_220000_Erzhausen/RConn3 -- L_160093341/LConn3
  T_43072656_220000;110000_Hardegsen/RConn1 -- L_43072656/LConn1
  T_43072656_220000;110000_Hardegsen/RConn2 -- L_43072656/LConn2
  T_43072656_220000;110000_Hardegsen/RConn3 -- L_43072656/LConn3
  T_30109913_220000;110000_Godenau/RConn1 -- L_30109913/LConn1
  T_30109913_220000;110000_Godenau/RConn2 -- L_30109913/LConn2
  T_30109913_220000;110000_Godenau/RConn3 -- L_30109913/LConn3
  T_202580524_380000_/RConn1 -- L_202580524/LConn1
  T_202580524_380000_/RConn2 -- L_202580524/LConn2
  T_202580524_380000_/RConn3 -- L_202580524/LConn3
  T_285823537__/RConn1 -- L_285823537/LConn1
  T_285823537__/RConn2 -- L_285823537/LConn2
  T_285823537__/RConn3 -- L_285823537/LConn3
  T_31019939_380000;110000_Gundremmingen/RConn1 -- L_31019939/LConn1
  T_31019939_380000;110000_Gundremmingen/RConn2 -- L_31019939/LConn2
  T_31019939_380000;110000_Gundremmingen/RConn3 -- L_31019939/LConn3
  T_266684854_380000_Umspannwerk_Farge/RConn1 -- L_266684854/LConn1
  T_266684854_380000_Umspannwerk_Farge/RConn2 -- L_266684854/LConn2
  T_266684854_380000_Umspannwerk_Farge/RConn3 -- L_266684854/LConn3
  T_22766160_380000;220000;110000_Station_Sechtem/RConn4 -- L_22766160/LConn1
  T_22766160_380000;220000;110000_Station_Sechtem/RConn5 -- L_22766160/LConn2
  T_22766160_380000;220000;110000_Station_Sechtem/RConn6 -- L_22766160/LConn3
  T_32148946_220000;110000_Station_Bollenacker/RConn1 -- L_32148946/LConn1
  T_32148946_220000;110000_Station_Bollenacker/RConn2 -- L_32148946/LConn2
  T_32148946_220000;110000_Station_Bollenacker/RConn3 -- L_32148946/LConn3
  T_23084554_220000;110000_Station_Brauweiler/RConn1 -- L_23084554/LConn1
  T_23084554_220000;110000_Station_Brauweiler/RConn2 -- L_23084554/LConn2
  T_23084554_220000;110000_Station_Brauweiler/RConn3 -- L_23084554/LConn3
  T_22765517_380000;110000_Station_Knapsack/RConn1 -- L_22765517/LConn1
  T_22765517_380000;110000_Station_Knapsack/RConn2 -- L_22765517/LConn2
  T_22765517_380000;110000_Station_Knapsack/RConn3 -- L_22765517/LConn3
  T_26777313_380000;110000_Station_Ließem/RConn1 -- L_26777313/LConn1
  T_26777313_380000;110000_Station_Ließem/RConn2 -- L_26777313/LConn2
  T_26777313_380000;110000_Station_Ließem/RConn3 -- L_26777313/LConn3
  T_26403575_380000;110000_EnBW_Umspannwerk_Bünzwangen/RConn1 -- L_26403575/LConn1
  T_26403575_380000;110000_EnBW_Umspannwerk_Bünzwangen/RConn2 -- L_26403575/LConn2
  T_26403575_380000;110000_EnBW_Umspannwerk_Bünzwangen/RConn3 -- L_26403575/LConn3
  T_30734324_380000;220000;110000_EnBW_Umspannwerk_Metzingen/RConn1 -- L_30734324/LConn1
  T_30734324_380000;220000;110000_EnBW_Umspannwerk_Metzingen/RConn2 -- L_30734324/LConn2
  T_30734324_380000;220000;110000_EnBW_Umspannwerk_Metzingen/RConn3 -- L_30734324/LConn3
  T_22960899_380000;110000_Umspannwerk_Mühlhausen/RConn1 -- L_22960899/LConn1
  T_22960899_380000;110000_Umspannwerk_Mühlhausen/RConn2 -- L_22960899/LConn2
  T_22960899_380000;110000_Umspannwerk_Mühlhausen/RConn3 -- L_22960899/LConn3
  T_59026005_380000;110000_Umspannwerk_Hagenwerder/RConn1 -- L_59026005/LConn1
  T_59026005_380000;110000_Umspannwerk_Hagenwerder/RConn2 -- L_59026005/LConn2
  T_59026005_380000;110000_Umspannwerk_Hagenwerder/RConn3 -- L_59026005/LConn3
  T_89043564_220000;110000_Station_Eiserfeld/RConn1 -- L_89043564/LConn1
  T_89043564_220000;110000_Station_Eiserfeld/RConn2 -- L_89043564/LConn2
  T_89043564_220000;110000_Station_Eiserfeld/RConn3 -- L_89043564/LConn3
  T_132814303_220000;110000_Station_Altenkleusheim/RConn1 -- L_132814303/LConn1
  T_132814303_220000;110000_Station_Altenkleusheim/RConn2 -- L_132814303/LConn2
  T_132814303_220000;110000_Station_Altenkleusheim/RConn3 -- L_132814303/LConn3
  T_26814283_380000;110000_EnBW_Umspannwerk_Oberjettingen/RConn1 -- L_26814283/LConn1
  T_26814283_380000;110000_EnBW_Umspannwerk_Oberjettingen/RConn2 -- L_26814283/LConn2
  T_26814283_380000;110000_EnBW_Umspannwerk_Oberjettingen/RConn3 -- L_26814283/LConn3
  T_23284340_380000;220000;110000_Umspannwerk_Urberach/RConn4 -- L_23284340/LConn1
  T_23284340_380000;220000;110000_Umspannwerk_Urberach/RConn5 -- L_23284340/LConn2
  T_23284340_380000;220000;110000_Umspannwerk_Urberach/RConn6 -- L_23284340/LConn3
  T_31718547__/RConn1 -- L_31718547/LConn1
  T_31718547__/RConn2 -- L_31718547/LConn2
  T_31718547__/RConn3 -- L_31718547/LConn3
  T_160533153_220000;110000_Beerfelden/RConn1 -- L_160533153/LConn1
  T_160533153_220000;110000_Beerfelden/RConn2 -- L_160533153/LConn2
  T_160533153_220000;110000_Beerfelden/RConn3 -- L_160533153/LConn3
  T_24685992_380000;110000_Umspannstation_Bischofsheim/RConn1 -- L_24685992/LConn1
  T_24685992_380000;110000_Umspannstation_Bischofsheim/RConn2 -- L_24685992/LConn2
  T_24685992_380000;110000_Umspannstation_Bischofsheim/RConn3 -- L_24685992/LConn3
  T_160584794_380000;110000_Station_Koblenz/RConn1 -- L_160584794/LConn1
  T_160584794_380000;110000_Station_Koblenz/RConn2 -- L_160584794/LConn2
  T_160584794_380000;110000_Station_Koblenz/RConn3 -- L_160584794/LConn3
  T_50898216_380000;110000_Station_Limburg/RConn1 -- L_50898216/LConn1
  T_50898216_380000;110000_Station_Limburg/RConn2 -- L_50898216/LConn2
  T_50898216_380000;110000_Station_Limburg/RConn3 -- L_50898216/LConn3
  T_38661452_380000;110000_Umspannwerk_Kriftel/RConn1 -- L_38661452/LConn1
  T_38661452_380000;110000_Umspannwerk_Kriftel/RConn2 -- L_38661452/LConn2
  T_38661452_380000;110000_Umspannwerk_Kriftel/RConn3 -- L_38661452/LConn3
  T_42372159_380000;110000_Karlstein/RConn1 -- L_42372159/LConn1
  T_42372159_380000;110000_Karlstein/RConn2 -- L_42372159/LConn2
  T_42372159_380000;110000_Karlstein/RConn3 -- L_42372159/LConn3
  T_274621059_220000;110000_Mehrum_(220_kV)/RConn1 -- L_274621059/LConn1
  T_274621059_220000;110000_Mehrum_(220_kV)/RConn2 -- L_274621059/LConn2
  T_274621059_220000;110000_Mehrum_(220_kV)/RConn3 -- L_274621059/LConn3
  T_46584363_380000;220000;110000_Umspannwerk_Wiesloch/RConn1 -- L_46584363/LConn1
  T_46584363_380000;220000;110000_Umspannwerk_Wiesloch/RConn2 -- L_46584363/LConn2
  T_46584363_380000;220000;110000_Umspannwerk_Wiesloch/RConn3 -- L_46584363/LConn3
  T_121199242_380000_Station_Lippe/RConn1 -- L_121199242/LConn1
  T_121199242_380000_Station_Lippe/RConn2 -- L_121199242/LConn2
  T_121199242_380000_Station_Lippe/RConn3 -- L_121199242/LConn3
  T_30954714_380000;110000_Umspannwerk_Friedrichshain/RConn1 -- L_30954714/LConn1
  T_30954714_380000;110000_Umspannwerk_Friedrichshain/RConn2 -- L_30954714/LConn2
  T_30954714_380000;110000_Umspannwerk_Friedrichshain/RConn3 -- L_30954714/LConn3
  T_26593935_380000_Station_Hambach/RConn1 -- L_26593935/LConn1
  T_26593935_380000_Station_Hambach/RConn2 -- L_26593935/LConn2
  T_26593935_380000_Station_Hambach/RConn3 -- L_26593935/LConn3
  T_27919734_220000;110000_Station_Gohrpunkt/RConn1 -- L_27919734/LConn1
  T_27919734_220000;110000_Station_Gohrpunkt/RConn2 -- L_27919734/LConn2
  T_27919734_220000;110000_Station_Gohrpunkt/RConn3 -- L_27919734/LConn3
  T_35818134_220000;110000_Station_Ruhrort/RConn1 -- L_35818134/LConn1
  T_35818134_220000;110000_Station_Ruhrort/RConn2 -- L_35818134/LConn2
  T_35818134_220000;110000_Station_Ruhrort/RConn3 -- L_35818134/LConn3
  T_35818522_220000_/RConn1 -- L_35818522/LConn1
  T_35818522_220000_/RConn2 -- L_35818522/LConn2
  T_35818522_220000_/RConn3 -- L_35818522/LConn3
  T_66038431_220000;110000_Station_Laer/RConn1 -- L_66038431/LConn1
  T_66038431_220000;110000_Station_Laer/RConn2 -- L_66038431/LConn2
  T_66038431_220000;110000_Station_Laer/RConn3 -- L_66038431/LConn3
  T_24667346_220000;110000_Umspannwerk_Garenfeld/RConn1 -- L_24667346/LConn1
  T_24667346_220000;110000_Umspannwerk_Garenfeld/RConn2 -- L_24667346/LConn2
  T_24667346_220000;110000_Umspannwerk_Garenfeld/RConn3 -- L_24667346/LConn3
  T_39688875_220000_Umspannwerk_Windpark_Iven/RConn1 -- L_39688875/LConn1
  T_39688875_220000_Umspannwerk_Windpark_Iven/RConn2 -- L_39688875/LConn2
  T_39688875_220000_Umspannwerk_Windpark_Iven/RConn3 -- L_39688875/LConn3
  T_39437430_220000;110000_Pasewalk/RConn1 -- L_39437430/LConn1
  T_39437430_220000;110000_Pasewalk/RConn2 -- L_39437430/LConn2
  T_39437430_220000;110000_Pasewalk/RConn3 -- L_39437430/LConn3
  T_32318130_220000;110000_Bentwisch/RConn1 -- L_32318130/LConn1
  T_32318130_220000;110000_Bentwisch/RConn2 -- L_32318130/LConn2
  T_32318130_220000;110000_Bentwisch/RConn3 -- L_32318130/LConn3
  T_29389718_220000;110000_Umspannwerk_Lüdershagen/RConn1 -- L_29389718/LConn1
  T_29389718_220000;110000_Umspannwerk_Lüdershagen/RConn2 -- L_29389718/LConn2
  T_29389718_220000;110000_Umspannwerk_Lüdershagen/RConn3 -- L_29389718/LConn3
  T_24765111_220000;110000_Umspannwerk_Trennfeld/RConn1 -- L_24765111/LConn1
  T_24765111_220000;110000_Umspannwerk_Trennfeld/RConn2 -- L_24765111/LConn2
  T_24765111_220000;110000_Umspannwerk_Trennfeld/RConn3 -- L_24765111/LConn3
  T_133349218_220000;110000_Umspannwerk_Ludersheim/RConn1 -- L_133349218/LConn1
  T_133349218_220000;110000_Umspannwerk_Ludersheim/RConn2 -- L_133349218/LConn2
  T_133349218_220000;110000_Umspannwerk_Ludersheim/RConn3 -- L_133349218/LConn3
  T_55069713_380000;220000;110000_Umspannwerk_Aschaffenburg/RConn4 -- L_55069713/LConn1
  T_55069713_380000;220000;110000_Umspannwerk_Aschaffenburg/RConn5 -- L_55069713/LConn2
  T_55069713_380000;220000;110000_Umspannwerk_Aschaffenburg/RConn6 -- L_55069713/LConn3
  T_109917397_380000_Freiberg_Nord_(380_kV)/RConn1 -- L_109917397/LConn1
  T_109917397_380000_Freiberg_Nord_(380_kV)/RConn2 -- L_109917397/LConn2
  T_109917397_380000_Freiberg_Nord_(380_kV)/RConn3 -- L_109917397/LConn3
  T_23241863_380000;110000_Umspannwerk_DD_Süd/RConn1 -- L_23241863/LConn1
  T_23241863_380000;110000_Umspannwerk_DD_Süd/RConn2 -- L_23241863/LConn2
  T_23241863_380000;110000_Umspannwerk_DD_Süd/RConn3 -- L_23241863/LConn3
  T_24230738_380000;110000_Eickum/RConn1 -- L_24230738/LConn1
  T_24230738_380000;110000_Eickum/RConn2 -- L_24230738/LConn2
  T_24230738_380000;110000_Eickum/RConn3 -- L_24230738/LConn3
  T_31762305_220000;110000_Station_Norf/RConn1 -- L_31762305/LConn1
  T_31762305_220000;110000_Station_Norf/RConn2 -- L_31762305/LConn2
  T_31762305_220000;110000_Station_Norf/RConn3 -- L_31762305/LConn3
  T_90109304_220000_UA_Dillinger_Hütte_Mitte/RConn1 -- L_90109304/LConn1
  T_90109304_220000_UA_Dillinger_Hütte_Mitte/RConn2 -- L_90109304/LConn2
  T_90109304_220000_UA_Dillinger_Hütte_Mitte/RConn3 -- L_90109304/LConn3
  T_24768051_380000;220000;110000_Ingolstadt/RConn4 -- L_24768051/LConn1
  T_24768051_380000;220000;110000_Ingolstadt/RConn5 -- L_24768051/LConn2
  T_24768051_380000;220000;110000_Ingolstadt/RConn6 -- L_24768051/LConn3
  T_31367936_220000;110000_Umspannwerk_Stockach/RConn1 -- L_31367936/LConn1
  T_31367936_220000;110000_Umspannwerk_Stockach/RConn2 -- L_31367936/LConn2
  T_31367936_220000;110000_Umspannwerk_Stockach/RConn3 -- L_31367936/LConn3
  T_102743264_220000;110000_Beuren/RConn1 -- L_102743264/LConn1
  T_102743264_220000;110000_Beuren/RConn2 -- L_102743264/LConn2
  T_102743264_220000;110000_Beuren/RConn3 -- L_102743264/LConn3
  T_31367937_220000;110000_Umspannwerk_Gurtweil/RConn1 -- L_31367937/LConn1
  T_31367937_220000;110000_Umspannwerk_Gurtweil/RConn2 -- L_31367937/LConn2
  T_31367937_220000;110000_Umspannwerk_Gurtweil/RConn3 -- L_31367937/LConn3
  T_77697810_380000_Isar/RConn1 -- L_77697810/LConn1
  T_77697810_380000_Isar/RConn2 -- L_77697810/LConn2
  T_77697810_380000_Isar/RConn3 -- L_77697810/LConn3
  T_51940126_220000;110000_Umspannwerk_Bixterheide/RConn1 -- L_51940126/LConn1
  T_51940126_220000;110000_Umspannwerk_Bixterheide/RConn2 -- L_51940126/LConn2
  T_51940126_220000;110000_Umspannwerk_Bixterheide/RConn3 -- L_51940126/LConn3
  T_272646943_380000_/RConn1 -- L_272646943/LConn1
  T_272646943_380000_/RConn2 -- L_272646943/LConn2
  T_272646943_380000_/RConn3 -- L_272646943/LConn3
  T_147878692_380000;110000_Umrichterwerk_Neckarwestheim/RConn1 -- L_147878692/LConn1
  T_147878692_380000;110000_Umrichterwerk_Neckarwestheim/RConn2 -- L_147878692/LConn2
  T_147878692_380000;110000_Umrichterwerk_Neckarwestheim/RConn3 -- L_147878692/LConn3
  T_118928165_220000_Benteler_Stahlwerk/RConn1 -- L_118928165/LConn1
  T_118928165_220000_Benteler_Stahlwerk/RConn2 -- L_118928165/LConn2
  T_118928165_220000_Benteler_Stahlwerk/RConn3 -- L_118928165/LConn3
  T_92877610__/RConn1 -- L_92877610/LConn1
  T_92877610__/RConn2 -- L_92877610/LConn2
  T_92877610__/RConn3 -- L_92877610/LConn3
  T_90807341_220000;110000_Umspannwerk_Kempten_Au/RConn1 -- L_90807341/LConn1
  T_90807341_220000;110000_Umspannwerk_Kempten_Au/RConn2 -- L_90807341/LConn2
  T_90807341_220000;110000_Umspannwerk_Kempten_Au/RConn3 -- L_90807341/LConn3
  T_23907283_380000;110000_Hauptumspannwerk_Menzing/RConn1 -- L_23907283/LConn1
  T_23907283_380000;110000_Hauptumspannwerk_Menzing/RConn2 -- L_23907283/LConn2
  T_23907283_380000;110000_Hauptumspannwerk_Menzing/RConn3 -- L_23907283/LConn3
  T_111973179_220000;110000_Station_Münster/RConn1 -- L_111973179/LConn1
  T_111973179_220000;110000_Station_Münster/RConn2 -- L_111973179/LConn2
  T_111973179_220000;110000_Station_Münster/RConn3 -- L_111973179/LConn3
  T_92877635__/RConn1 -- L_92877635/LConn1
  T_92877635__/RConn2 -- L_92877635/LConn2
  T_92877635__/RConn3 -- L_92877635/LConn3
  T_28327356_380000;110000_Lüneburg/RConn1 -- L_28327356/LConn1
  T_28327356_380000;110000_Lüneburg/RConn2 -- L_28327356/LConn2
  T_28327356_380000;110000_Lüneburg/RConn3 -- L_28327356/LConn3
  T_60032354_220000;110000_Itzehoe_West/RConn1 -- L_60032354/LConn1
  T_60032354_220000;110000_Itzehoe_West/RConn2 -- L_60032354/LConn2
  T_60032354_220000;110000_Itzehoe_West/RConn3 -- L_60032354/LConn3
  T_156673636_380000;110000_Umspannwerk_Borken/RConn1 -- L_156673636/LConn1
  T_156673636_380000;110000_Umspannwerk_Borken/RConn2 -- L_156673636/LConn2
  T_156673636_380000;110000_Umspannwerk_Borken/RConn3 -- L_156673636/LConn3
  T_148446247_380000;110000_UW_Dipperz/RConn1 -- L_148446247/LConn1
  T_148446247_380000;110000_UW_Dipperz/RConn2 -- L_148446247/LConn2
  T_148446247_380000;110000_UW_Dipperz/RConn3 -- L_148446247/LConn3
  T_232833796_220000_/RConn1 -- L_232833796/LConn1
  T_232833796_220000_/RConn2 -- L_232833796/LConn2
  T_232833796_220000_/RConn3 -- L_232833796/LConn3
  T_29103809_220000;110000_Umspannwerk_Rosdorf/RConn1 -- L_29103809/LConn1
  T_29103809_220000;110000_Umspannwerk_Rosdorf/RConn2 -- L_29103809/LConn2
  T_29103809_220000;110000_Umspannwerk_Rosdorf/RConn3 -- L_29103809/LConn3
  T_254326606_380000;110000_Umspannwerk_Bruchsal_Kändelweg/RConn1 -- L_254326606/LConn1
  T_254326606_380000;110000_Umspannwerk_Bruchsal_Kändelweg/RConn2 -- L_254326606/LConn2
  T_254326606_380000;110000_Umspannwerk_Bruchsal_Kändelweg/RConn3 -- L_254326606/LConn3
  T_89176939_220000_SA_Bauler/RConn1 -- L_89176939/LConn1
  T_89176939_220000_SA_Bauler/RConn2 -- L_89176939/LConn2
  T_89176939_220000_SA_Bauler/RConn3 -- L_89176939/LConn3
  T_89176956_220000_Vianden/RConn1 -- L_89176956/LConn1
  T_89176956_220000_Vianden/RConn2 -- L_89176956/LConn2
  T_89176956_220000_Vianden/RConn3 -- L_89176956/LConn3
  T_39428980_220000;110000_Vierraden/RConn1 -- L_39428980/LConn1
  T_39428980_220000;110000_Vierraden/RConn2 -- L_39428980/LConn2
  T_39428980_220000;110000_Vierraden/RConn3 -- L_39428980/LConn3
  T_30039908_380000;220000_Bertikow/RConn1 -- L_30039908/LConn1
  T_30039908_380000;220000_Bertikow/RConn2 -- L_30039908/LConn2
  T_30039908_380000;220000_Bertikow/RConn3 -- L_30039908/LConn3
  T_24042358_380000;110000_Umspannwerk_Karben/RConn1 -- L_24042358/LConn1
  T_24042358_380000;110000_Umspannwerk_Karben/RConn2 -- L_24042358/LConn2
  T_24042358_380000;110000_Umspannwerk_Karben/RConn3 -- L_24042358/LConn3
  T_202747445_380000;110000_Umspannwerk_Gießen_Nord/RConn1 -- L_202747445/LConn1
  T_202747445_380000;110000_Umspannwerk_Gießen_Nord/RConn2 -- L_202747445/LConn2
  T_202747445_380000;110000_Umspannwerk_Gießen_Nord/RConn3 -- L_202747445/LConn3
  T_62061952_380000_Umspannwerk_Frankfurt_Südwest/RConn1 -- L_62061952/LConn1
  T_62061952_380000_Umspannwerk_Frankfurt_Südwest/RConn2 -- L_62061952/LConn2
  T_62061952_380000_Umspannwerk_Frankfurt_Südwest/RConn3 -- L_62061952/LConn3
  T_172997498_220000;110000_Sandershausen/RConn1 -- L_172997498/LConn1
  T_172997498_220000;110000_Sandershausen/RConn2 -- L_172997498/LConn2
  T_172997498_220000;110000_Sandershausen/RConn3 -- L_172997498/LConn3
  T_274630377_380000;220000;110000_Umspannanlage_Würgassen/RConn4 -- L_274630377/LConn1
  T_274630377_380000;220000;110000_Umspannanlage_Würgassen/RConn5 -- L_274630377/LConn2
  T_274630377_380000;220000;110000_Umspannanlage_Würgassen/RConn6 -- L_274630377/LConn3
  T_27124619_220000;110000_Kiel_Süd/RConn1 -- L_27124619/LConn1
  T_27124619_220000;110000_Kiel_Süd/RConn2 -- L_27124619/LConn2
  T_27124619_220000;110000_Kiel_Süd/RConn3 -- L_27124619/LConn3
  T_33148774_220000;110000_Audorf/RConn1 -- L_33148774/LConn1
  T_33148774_220000;110000_Audorf/RConn2 -- L_33148774/LConn2
  T_33148774_220000;110000_Audorf/RConn3 -- L_33148774/LConn3
  T_27646106_220000;110000_Umspannwerk_Kiel_West/RConn1 -- L_27646106/LConn1
  T_27646106_220000;110000_Umspannwerk_Kiel_West/RConn2 -- L_27646106/LConn2
  T_27646106_220000;110000_Umspannwerk_Kiel_West/RConn3 -- L_27646106/LConn3
  T_59925390_380000;110000_Station_Karnap/RConn1 -- L_59925390/LConn1
  T_59925390_380000;110000_Station_Karnap/RConn2 -- L_59925390/LConn2
  T_59925390_380000;110000_Station_Karnap/RConn3 -- L_59925390/LConn3
  T_193674783__/RConn1 -- L_193674783/LConn1
  T_193674783__/RConn2 -- L_193674783/LConn2
  T_193674783__/RConn3 -- L_193674783/LConn3
  T_173112252_220000;110000_Crossen/RConn1 -- L_173112252/LConn1
  T_173112252_220000;110000_Crossen/RConn2 -- L_173112252/LConn2
  T_173112252_220000;110000_Crossen/RConn3 -- L_173112252/LConn3
  T_32076853_380000;220000;110000_Unterweser/RConn4 -- L_32076853/LConn1
  T_32076853_380000;220000;110000_Unterweser/RConn5 -- L_32076853/LConn2
  T_32076853_380000;220000;110000_Unterweser/RConn6 -- L_32076853/LConn3
  T_32725958_220000;110000_Karlsruhe_Rintheim/RConn1 -- L_32725958/LConn1
  T_32725958_220000;110000_Karlsruhe_Rintheim/RConn2 -- L_32725958/LConn2
  T_32725958_220000;110000_Karlsruhe_Rintheim/RConn3 -- L_32725958/LConn3
  T_23682013_220000;110000_Hannover_West/RConn1 -- L_23682013/LConn1
  T_23682013_220000;110000_Hannover_West/RConn2 -- L_23682013/LConn2
  T_23682013_220000;110000_Hannover_West/RConn3 -- L_23682013/LConn3
  T_44717036_380000;110000_Niedervieland/RConn1 -- L_44717036/LConn1
  T_44717036_380000;110000_Niedervieland/RConn2 -- L_44717036/LConn2
  T_44717036_380000;110000_Niedervieland/RConn3 -- L_44717036/LConn3
  T_24493551_380000;110000_Ganderkesee/RConn1 -- L_24493551/LConn1
  T_24493551_380000;110000_Ganderkesee/RConn2 -- L_24493551/LConn2
  T_24493551_380000;110000_Ganderkesee/RConn3 -- L_24493551/LConn3
  T_40621568_220000;110000_Brandenburg_West/RConn1 -- L_40621568/LConn1
  T_40621568_220000;110000_Brandenburg_West/RConn2 -- L_40621568/LConn2
  T_40621568_220000;110000_Brandenburg_West/RConn3 -- L_40621568/LConn3
  T_194446360_380000_/RConn1 -- L_194446360/LConn1
  T_194446360_380000_/RConn2 -- L_194446360/LConn2
  T_194446360_380000_/RConn3 -- L_194446360/LConn3
  T_24759324_220000;110000_Umspannwerk_Sittling/RConn1 -- L_24759324/LConn1
  T_24759324_220000;110000_Umspannwerk_Sittling/RConn2 -- L_24759324/LConn2
  T_24759324_220000;110000_Umspannwerk_Sittling/RConn3 -- L_24759324/LConn3
  T_22690852_220000;110000_Bocklemünd/RConn1 -- L_22690852/LConn1
  T_22690852_220000;110000_Bocklemünd/RConn2 -- L_22690852/LConn2
  T_22690852_220000;110000_Bocklemünd/RConn3 -- L_22690852/LConn3
  T_109582315_380000;220000_Kernkraftwerk_Unterweser/RConn1 -- L_109582315/LConn1
  T_109582315_380000;220000_Kernkraftwerk_Unterweser/RConn2 -- L_109582315/LConn2
  T_109582315_380000;220000_Kernkraftwerk_Unterweser/RConn3 -- L_109582315/LConn3
  T_11500045_380000_380_kV_Kabel_Terminal_Berlin/RConn1 -- L_11500045/LConn1
  T_11500045_380000_380_kV_Kabel_Terminal_Berlin/RConn2 -- L_11500045/LConn2
  T_11500045_380000_380_kV_Kabel_Terminal_Berlin/RConn3 -- L_11500045/LConn3
  T_46615737_380000;110000_Umspannwerk_Charlottenburg/RConn1 -- L_46615737/LConn1
  T_46615737_380000;110000_Umspannwerk_Charlottenburg/RConn2 -- L_46615737/LConn2
  T_46615737_380000;110000_Umspannwerk_Charlottenburg/RConn3 -- L_46615737/LConn3
  T_176704629__/RConn1 -- L_176704629/LConn1
  T_176704629__/RConn2 -- L_176704629/LConn2
  T_176704629__/RConn3 -- L_176704629/LConn3
  T_150267232_220000_LMG/RConn1 -- L_150267232/LConn1
  T_150267232_220000_LMG/RConn2 -- L_150267232/LConn2
  T_150267232_220000_LMG/RConn3 -- L_150267232/LConn3
  T_42423415_220000;110000_Station_Meckenheim/RConn1 -- L_42423415/LConn1
  T_42423415_220000;110000_Station_Meckenheim/RConn2 -- L_42423415/LConn2
  T_42423415_220000;110000_Station_Meckenheim/RConn3 -- L_42423415/LConn3
  T_42681484_380000;110000_Vörden/RConn1 -- L_42681484/LConn1
  T_42681484_380000;110000_Vörden/RConn2 -- L_42681484/LConn2
  T_42681484_380000;110000_Vörden/RConn3 -- L_42681484/LConn3
  T_152219167_220000_Stahlwerk_Thüringen/RConn1 -- L_152219167/LConn1
  T_152219167_220000_Stahlwerk_Thüringen/RConn2 -- L_152219167/LConn2
  T_152219167_220000_Stahlwerk_Thüringen/RConn3 -- L_152219167/LConn3
  T_156673637_380000;220000;110000_Umspannwerk_Weida/RConn4 -- L_156673637/LConn1
  T_156673637_380000;220000;110000_Umspannwerk_Weida/RConn5 -- L_156673637/LConn2
  T_156673637_380000;220000;110000_Umspannwerk_Weida/RConn6 -- L_156673637/LConn3
  T_24536211_380000;110000_Umspannwerk_Aßlar/RConn1 -- L_24536211/LConn1
  T_24536211_380000;110000_Umspannwerk_Aßlar/RConn2 -- L_24536211/LConn2
  T_24536211_380000;110000_Umspannwerk_Aßlar/RConn3 -- L_24536211/LConn3
  T_24536328_380000;110000_Dillenburg/RConn1 -- L_24536328/LConn1
  T_24536328_380000;110000_Dillenburg/RConn2 -- L_24536328/LConn2
  T_24536328_380000;110000_Dillenburg/RConn3 -- L_24536328/LConn3
  T_23161029_220000;110000_Umspannwerk_Taucha/RConn1 -- L_23161029/LConn1
  T_23161029_220000;110000_Umspannwerk_Taucha/RConn2 -- L_23161029/LConn2
  T_23161029_220000;110000_Umspannwerk_Taucha/RConn3 -- L_23161029/LConn3
  T_24478889_220000;110000_Station_Walsum/RConn1 -- L_24478889/LConn1
  T_24478889_220000;110000_Station_Walsum/RConn2 -- L_24478889/LConn2
  T_24478889_220000;110000_Station_Walsum/RConn3 -- L_24478889/LConn3
  T_30303506_380000;110000_Berlin_Mitte/RConn1 -- L_30303506/LConn1
  T_30303506_380000;110000_Berlin_Mitte/RConn2 -- L_30303506/LConn2
  T_30303506_380000;110000_Berlin_Mitte/RConn3 -- L_30303506/LConn3
  T_83916207_220000;110000_Elverlingsen/RConn1 -- L_83916207/LConn1
  T_83916207_220000;110000_Elverlingsen/RConn2 -- L_83916207/LConn2
  T_83916207_220000;110000_Elverlingsen/RConn3 -- L_83916207/LConn3
  T_100812630_220000;110000_/RConn1 -- L_100812630/LConn1
  T_100812630_220000;110000_/RConn2 -- L_100812630/LConn2
  T_100812630_220000;110000_/RConn3 -- L_100812630/LConn3
  T_30309989_220000_Hennigsdorf/RConn1 -- L_30309989/LConn1
  T_30309989_220000_Hennigsdorf/RConn2 -- L_30309989/LConn2
  T_30309989_220000_Hennigsdorf/RConn3 -- L_30309989/LConn3
  T_35763481_380000;110000_Station_Witten/RConn1 -- L_35763481/LConn1
  T_35763481_380000;110000_Station_Witten/RConn2 -- L_35763481/LConn2
  T_35763481_380000;110000_Station_Witten/RConn3 -- L_35763481/LConn3
  T_24479003_220000_Station_Möllen/RConn4 -- L_24479003/LConn1
  T_24479003_220000_Station_Möllen/RConn5 -- L_24479003/LConn2
  T_24479003_220000_Station_Möllen/RConn6 -- L_24479003/LConn3
  T_29420322_220000;155000_Inhausen/RConn1 -- L_29420322/LConn1
  T_29420322_220000;155000_Inhausen/RConn2 -- L_29420322/LConn2
  T_29420322_220000;155000_Inhausen/RConn3 -- L_29420322/LConn3
  T_26455019_220000;110000_Voslapp/RConn1 -- L_26455019/LConn1
  T_26455019_220000;110000_Voslapp/RConn2 -- L_26455019/LConn2
  T_26455019_220000;110000_Voslapp/RConn3 -- L_26455019/LConn3
  T_48428875_380000;110000_EnBW_Umspannwerk_Endersbach/RConn1 -- L_48428875/LConn1
  T_48428875_380000;110000_EnBW_Umspannwerk_Endersbach/RConn2 -- L_48428875/LConn2
  T_48428875_380000;110000_EnBW_Umspannwerk_Endersbach/RConn3 -- L_48428875/LConn3
  T_156676050_220000;110000_Umspannanlage_Heidelberg_Süd/RConn1 -- L_156676050/LConn1
  T_156676050_220000;110000_Umspannanlage_Heidelberg_Süd/RConn2 -- L_156676050/LConn2
  T_156676050_220000;110000_Umspannanlage_Heidelberg_Süd/RConn3 -- L_156676050/LConn3
  T_76185022_380000_Station_Zensenbusch/RConn1 -- L_76185022/LConn1
  T_76185022_380000_Station_Zensenbusch/RConn2 -- L_76185022/LConn2
  T_76185022_380000_Station_Zensenbusch/RConn3 -- L_76185022/LConn3
  T_37721677_380000;110000_EnBW_Umspannwerk_Altbach_1/RConn1 -- L_37721677/LConn1
  T_37721677_380000;110000_EnBW_Umspannwerk_Altbach_1/RConn2 -- L_37721677/LConn2
  T_37721677_380000;110000_EnBW_Umspannwerk_Altbach_1/RConn3 -- L_37721677/LConn3
  T_43163132_380000;110000_Umspannwerk_Reuter/RConn1 -- L_43163132/LConn1
  T_43163132_380000;110000_Umspannwerk_Reuter/RConn2 -- L_43163132/LConn2
  T_43163132_380000;110000_Umspannwerk_Reuter/RConn3 -- L_43163132/LConn3
  T_154869247_220000_/RConn1 -- L_154869247/LConn1
  T_154869247_220000_/RConn2 -- L_154869247/LConn2
  T_154869247_220000_/RConn3 -- L_154869247/LConn3
  T_28921360_220000_Umspannwerk_Kraftwerk_Robert_Frank/RConn1 -- L_28921360/LConn1
  T_28921360_220000_Umspannwerk_Kraftwerk_Robert_Frank/RConn2 -- L_28921360/LConn2
  T_28921360_220000_Umspannwerk_Kraftwerk_Robert_Frank/RConn3 -- L_28921360/LConn3
  T_31131320_380000_Umspannwerk_Obermooweiler/RConn1 -- L_31131320/LConn1
  T_31131320_380000_Umspannwerk_Obermooweiler/RConn2 -- L_31131320/LConn2
  T_31131320_380000_Umspannwerk_Obermooweiler/RConn3 -- L_31131320/LConn3
  T_97857512_220000_/RConn1 -- L_97857512/LConn1
  T_97857512_220000_/RConn2 -- L_97857512/LConn2
  T_97857512_220000_/RConn3 -- L_97857512/LConn3
  T_42872354_220000_Huntorf/RConn1 -- L_42872354/LConn1
  T_42872354_220000_Huntorf/RConn2 -- L_42872354/LConn2
  T_42872354_220000_Huntorf/RConn3 -- L_42872354/LConn3
  T_23881272_220000;110000_Dörnigheim_220_kV/RConn1 -- L_23881272/LConn1
  T_23881272_220000;110000_Dörnigheim_220_kV/RConn2 -- L_23881272/LConn2
  T_23881272_220000;110000_Dörnigheim_220_kV/RConn3 -- L_23881272/LConn3
  T_4826893_220000;110000_Umspannwerk_Frankfurt_Nord/RConn1 -- L_4826893/LConn1
  T_4826893_220000;110000_Umspannwerk_Frankfurt_Nord/RConn2 -- L_4826893/LConn2
  T_4826893_220000;110000_Umspannwerk_Frankfurt_Nord/RConn3 -- L_4826893/LConn3
  T_32675761_380000;110000_Station_Dahlem/RConn1 -- L_32675761/LConn1
  T_32675761_380000;110000_Station_Dahlem/RConn2 -- L_32675761/LConn2
  T_32675761_380000;110000_Station_Dahlem/RConn3 -- L_32675761/LConn3
  T_167352587_220000;110000_Umspannwerk_Herlasgrün/RConn1 -- L_167352587/LConn1
  T_167352587_220000;110000_Umspannwerk_Herlasgrün/RConn2 -- L_167352587/LConn2
  T_167352587_220000;110000_Umspannwerk_Herlasgrün/RConn3 -- L_167352587/LConn3
  T_156960655_380000;110000_Umspannwerk_Bergshausen/RConn1 -- L_156960655/LConn1
  T_156960655_380000;110000_Umspannwerk_Bergshausen/RConn2 -- L_156960655/LConn2
  T_156960655_380000;110000_Umspannwerk_Bergshausen/RConn3 -- L_156960655/LConn3
  T_41072584_380000_UW_Waldeck/RConn1 -- L_41072584/LConn1
  T_41072584_380000_UW_Waldeck/RConn2 -- L_41072584/LConn2
  T_41072584_380000_UW_Waldeck/RConn3 -- L_41072584/LConn3
  T_106976898_220000_Saarstahl/RConn1 -- L_106976898/LConn1
  T_106976898_220000_Saarstahl/RConn2 -- L_106976898/LConn2
  T_106976898_220000_Saarstahl/RConn3 -- L_106976898/LConn3
  T_31135714_220000;110000_Umspannwerk_Heinitz/RConn1 -- L_31135714/LConn1
  T_31135714_220000;110000_Umspannwerk_Heinitz/RConn2 -- L_31135714/LConn2
  T_31135714_220000;110000_Umspannwerk_Heinitz/RConn3 -- L_31135714/LConn3
  T_25992879_380000;110000_Siersdorf/RConn1 -- L_25992879/LConn1
  T_25992879_380000;110000_Siersdorf/RConn2 -- L_25992879/LConn2
  T_25992879_380000;110000_Siersdorf/RConn3 -- L_25992879/LConn3
  T_23744346_380000;220000_Umspannwerk_Maade/RConn1 -- L_23744346/LConn1
  T_23744346_380000;220000_Umspannwerk_Maade/RConn2 -- L_23744346/LConn2
  T_23744346_380000;220000_Umspannwerk_Maade/RConn3 -- L_23744346/LConn3
  T_157449983_380000_/RConn1 -- L_157449983/LConn1
  T_157449983_380000_/RConn2 -- L_157449983/LConn2
  T_157449983_380000_/RConn3 -- L_157449983/LConn3
  T_157421330_220000_Atlantic/RConn1 -- L_157421330/LConn1
  T_157421330_220000_Atlantic/RConn2 -- L_157421330/LConn2
  T_157421330_220000_Atlantic/RConn3 -- L_157421330/LConn3
  T_82773910_380000;220000;110000_Umspannanlage_Ensdorf/RConn4 -- L_82773910/LConn1
  T_82773910_380000;220000;110000_Umspannanlage_Ensdorf/RConn5 -- L_82773910/LConn2
  T_82773910_380000;220000;110000_Umspannanlage_Ensdorf/RConn6 -- L_82773910/LConn3
  T_42411962_220000;110000_Kraftwerkseinspeisung_Staudinger/RConn1 -- L_42411962/LConn1
  T_42411962_220000;110000_Kraftwerkseinspeisung_Staudinger/RConn2 -- L_42411962/LConn2
  T_42411962_220000;110000_Kraftwerkseinspeisung_Staudinger/RConn3 -- L_42411962/LConn3
  T_23816140_220000;110000_Lahe/RConn1 -- L_23816140/LConn1
  T_23816140_220000;110000_Lahe/RConn2 -- L_23816140/LConn2
  T_23816140_220000;110000_Lahe/RConn3 -- L_23816140/LConn3
  T_275138524_380000;110000_Schaltanlage_Datteln_4/RConn1 -- L_275138524/LConn1
  T_275138524_380000;110000_Schaltanlage_Datteln_4/RConn2 -- L_275138524/LConn2
  T_275138524_380000;110000_Schaltanlage_Datteln_4/RConn3 -- L_275138524/LConn3
